simulink model "gm_minutiaeextraction_21821"  (R2018b)
(part 6 of 7)

  t38/53 -> concatenate/4789
  t38/54 -> concatenate/4790
  t38/55 -> concatenate/4791
  t38/56 -> concatenate/4792
  t38/57 -> concatenate/4793
  t38/58 -> concatenate/4794
  t38/59 -> concatenate/4795
  t38/60 -> concatenate/4796
  t38/61 -> concatenate/4797
  t38/62 -> concatenate/4798
  t38/63 -> concatenate/4799
  t38/64 -> concatenate/4800
  t38/65 -> concatenate/4801
  t38/66 -> concatenate/4802
  t38/67 -> concatenate/4803
  t38/68 -> concatenate/4804
  t38/69 -> concatenate/4805
  t38/70 -> concatenate/4806
  t38/71 -> concatenate/4807
  t38/72 -> concatenate/4808
  t38/73 -> concatenate/4809
  t38/74 -> concatenate/4810
  t38/75 -> concatenate/4811
  t38/76 -> concatenate/4812
  t38/77 -> concatenate/4813
  t38/78 -> concatenate/4814
  t38/79 -> concatenate/4815
  t38/80 -> concatenate/4816
  t38/81 -> concatenate/4817
  t38/82 -> concatenate/4818
  t38/83 -> concatenate/4819
  t38/84 -> concatenate/4820
  t38/85 -> concatenate/4821
  t38/86 -> concatenate/4822
  t38/87 -> concatenate/4823
  t38/88 -> concatenate/4824
  t38/89 -> concatenate/4825
  t38/90 -> concatenate/4826
  t38/91 -> concatenate/4827
  t38/92 -> concatenate/4828
  t38/93 -> concatenate/4829
  t38/94 -> concatenate/4830
  t38/95 -> concatenate/4831
  t38/96 -> concatenate/4832
  t38/97 -> concatenate/4833
  t38/98 -> concatenate/4834
  t38/99 -> concatenate/4835
  t38/100 -> concatenate/4836
  t38/101 -> concatenate/4837
  t38/102 -> concatenate/4838
  t38/103 -> concatenate/4839
  t38/104 -> concatenate/4840
  t38/105 -> concatenate/4841
  t38/106 -> concatenate/4842
  t38/107 -> concatenate/4843
  t38/108 -> concatenate/4844
  t38/109 -> concatenate/4845
  t38/110 -> concatenate/4846
  t38/111 -> concatenate/4847
  t38/112 -> concatenate/4848
  t38/113 -> concatenate/4849
  t38/114 -> concatenate/4850
  t38/115 -> concatenate/4851
  t38/116 -> concatenate/4852
  t38/117 -> concatenate/4853
  t38/118 -> concatenate/4854
  t38/119 -> concatenate/4855
  t38/120 -> concatenate/4856
  t38/121 -> concatenate/4857
  t38/122 -> concatenate/4858
  t38/123 -> concatenate/4859
  t38/124 -> concatenate/4860
  t38/125 -> concatenate/4861
  t38/126 -> concatenate/4862
  t38/127 -> concatenate/4863
  t38/128 -> concatenate/4864
  t39/1 -> concatenate/4865
  t39/2 -> concatenate/4866
  t39/3 -> concatenate/4867
  t39/4 -> concatenate/4868
  t39/5 -> concatenate/4869
  t39/6 -> concatenate/4870
  t39/7 -> concatenate/4871
  t39/8 -> concatenate/4872
  t39/9 -> concatenate/4873
  t39/10 -> concatenate/4874
  t39/11 -> concatenate/4875
  t39/12 -> concatenate/4876
  t39/13 -> concatenate/4877
  t39/14 -> concatenate/4878
  t39/15 -> concatenate/4879
  t39/16 -> concatenate/4880
  t39/17 -> concatenate/4881
  t39/18 -> concatenate/4882
  t39/19 -> concatenate/4883
  t39/20 -> concatenate/4884
  t39/21 -> concatenate/4885
  t39/22 -> concatenate/4886
  t39/23 -> concatenate/4887
  t39/24 -> concatenate/4888
  t39/25 -> concatenate/4889
  t39/26 -> concatenate/4890
  t39/27 -> concatenate/4891
  t39/28 -> concatenate/4892
  t39/29 -> concatenate/4893
  t39/30 -> concatenate/4894
  t39/31 -> concatenate/4895
  t39/32 -> concatenate/4896
  t39/33 -> concatenate/4897
  t39/34 -> concatenate/4898
  t39/35 -> concatenate/4899
  t39/36 -> concatenate/4900
  t39/37 -> concatenate/4901
  t39/38 -> concatenate/4902
  t39/39 -> concatenate/4903
  t39/40 -> concatenate/4904
  t39/41 -> concatenate/4905
  t39/42 -> concatenate/4906
  t39/43 -> concatenate/4907
  t39/44 -> concatenate/4908
  t39/45 -> concatenate/4909
  t39/46 -> concatenate/4910
  t39/47 -> concatenate/4911
  t39/48 -> concatenate/4912
  t39/49 -> concatenate/4913
  t39/50 -> concatenate/4914
  t39/51 -> concatenate/4915
  t39/52 -> concatenate/4916
  t39/53 -> concatenate/4917
  t39/54 -> concatenate/4918
  t39/55 -> concatenate/4919
  t39/56 -> concatenate/4920
  t39/57 -> concatenate/4921
  t39/58 -> concatenate/4922
  t39/59 -> concatenate/4923
  t39/60 -> concatenate/4924
  t39/61 -> concatenate/4925
  t39/62 -> concatenate/4926
  t39/63 -> concatenate/4927
  t39/64 -> concatenate/4928
  t39/65 -> concatenate/4929
  t39/66 -> concatenate/4930
  t39/67 -> concatenate/4931
  t39/68 -> concatenate/4932
  t39/69 -> concatenate/4933
  t39/70 -> concatenate/4934
  t39/71 -> concatenate/4935
  t39/72 -> concatenate/4936
  t39/73 -> concatenate/4937
  t39/74 -> concatenate/4938
  t39/75 -> concatenate/4939
  t39/76 -> concatenate/4940
  t39/77 -> concatenate/4941
  t39/78 -> concatenate/4942
  t39/79 -> concatenate/4943
  t39/80 -> concatenate/4944
  t39/81 -> concatenate/4945
  t39/82 -> concatenate/4946
  t39/83 -> concatenate/4947
  t39/84 -> concatenate/4948
  t39/85 -> concatenate/4949
  t39/86 -> concatenate/4950
  t39/87 -> concatenate/4951
  t39/88 -> concatenate/4952
  t39/89 -> concatenate/4953
  t39/90 -> concatenate/4954
  t39/91 -> concatenate/4955
  t39/92 -> concatenate/4956
  t39/93 -> concatenate/4957
  t39/94 -> concatenate/4958
  t39/95 -> concatenate/4959
  t39/96 -> concatenate/4960
  t39/97 -> concatenate/4961
  t39/98 -> concatenate/4962
  t39/99 -> concatenate/4963
  t39/100 -> concatenate/4964
  t39/101 -> concatenate/4965
  t39/102 -> concatenate/4966
  t39/103 -> concatenate/4967
  t39/104 -> concatenate/4968
  t39/105 -> concatenate/4969
  t39/106 -> concatenate/4970
  t39/107 -> concatenate/4971
  t39/108 -> concatenate/4972
  t39/109 -> concatenate/4973
  t39/110 -> concatenate/4974
  t39/111 -> concatenate/4975
  t39/112 -> concatenate/4976
  t39/113 -> concatenate/4977
  t39/114 -> concatenate/4978
  t39/115 -> concatenate/4979
  t39/116 -> concatenate/4980
  t39/117 -> concatenate/4981
  t39/118 -> concatenate/4982
  t39/119 -> concatenate/4983
  t39/120 -> concatenate/4984
  t39/121 -> concatenate/4985
  t39/122 -> concatenate/4986
  t39/123 -> concatenate/4987
  t39/124 -> concatenate/4988
  t39/125 -> concatenate/4989
  t39/126 -> concatenate/4990
  t39/127 -> concatenate/4991
  t39/128 -> concatenate/4992
  t40/1 -> concatenate/4993
  t40/2 -> concatenate/4994
  t40/3 -> concatenate/4995
  t40/4 -> concatenate/4996
  t40/5 -> concatenate/4997
  t40/6 -> concatenate/4998
  t40/7 -> concatenate/4999
  t40/8 -> concatenate/5000
  t40/9 -> concatenate/5001
  t40/10 -> concatenate/5002
  t40/11 -> concatenate/5003
  t40/12 -> concatenate/5004
  t40/13 -> concatenate/5005
  t40/14 -> concatenate/5006
  t40/15 -> concatenate/5007
  t40/16 -> concatenate/5008
  t40/17 -> concatenate/5009
  t40/18 -> concatenate/5010
  t40/19 -> concatenate/5011
  t40/20 -> concatenate/5012
  t40/21 -> concatenate/5013
  t40/22 -> concatenate/5014
  t40/23 -> concatenate/5015
  t40/24 -> concatenate/5016
  t40/25 -> concatenate/5017
  t40/26 -> concatenate/5018
  t40/27 -> concatenate/5019
  t40/28 -> concatenate/5020
  t40/29 -> concatenate/5021
  t40/30 -> concatenate/5022
  t40/31 -> concatenate/5023
  t40/32 -> concatenate/5024
  t40/33 -> concatenate/5025
  t40/34 -> concatenate/5026
  t40/35 -> concatenate/5027
  t40/36 -> concatenate/5028
  t40/37 -> concatenate/5029
  t40/38 -> concatenate/5030
  t40/39 -> concatenate/5031
  t40/40 -> concatenate/5032
  t40/41 -> concatenate/5033
  t40/42 -> concatenate/5034
  t40/43 -> concatenate/5035
  t40/44 -> concatenate/5036
  t40/45 -> concatenate/5037
  t40/46 -> concatenate/5038
  t40/47 -> concatenate/5039
  t40/48 -> concatenate/5040
  t40/49 -> concatenate/5041
  t40/50 -> concatenate/5042
  t40/51 -> concatenate/5043
  t40/52 -> concatenate/5044
  t40/53 -> concatenate/5045
  t40/54 -> concatenate/5046
  t40/55 -> concatenate/5047
  t40/56 -> concatenate/5048
  t40/57 -> concatenate/5049
  t40/58 -> concatenate/5050
  t40/59 -> concatenate/5051
  t40/60 -> concatenate/5052
  t40/61 -> concatenate/5053
  t40/62 -> concatenate/5054
  t40/63 -> concatenate/5055
  t40/64 -> concatenate/5056
  t40/65 -> concatenate/5057
  t40/66 -> concatenate/5058
  t40/67 -> concatenate/5059
  t40/68 -> concatenate/5060
  t40/69 -> concatenate/5061
  t40/70 -> concatenate/5062
  t40/71 -> concatenate/5063
  t40/72 -> concatenate/5064
  t40/73 -> concatenate/5065
  t40/74 -> concatenate/5066
  t40/75 -> concatenate/5067
  t40/76 -> concatenate/5068
  t40/77 -> concatenate/5069
  t40/78 -> concatenate/5070
  t40/79 -> concatenate/5071
  t40/80 -> concatenate/5072
  t40/81 -> concatenate/5073
  t40/82 -> concatenate/5074
  t40/83 -> concatenate/5075
  t40/84 -> concatenate/5076
  t40/85 -> concatenate/5077
  t40/86 -> concatenate/5078
  t40/87 -> concatenate/5079
  t40/88 -> concatenate/5080
  t40/89 -> concatenate/5081
  t40/90 -> concatenate/5082
  t40/91 -> concatenate/5083
  t40/92 -> concatenate/5084
  t40/93 -> concatenate/5085
  t40/94 -> concatenate/5086
  t40/95 -> concatenate/5087
  t40/96 -> concatenate/5088
  t40/97 -> concatenate/5089
  t40/98 -> concatenate/5090
  t40/99 -> concatenate/5091
  t40/100 -> concatenate/5092
  t40/101 -> concatenate/5093
  t40/102 -> concatenate/5094
  t40/103 -> concatenate/5095
  t40/104 -> concatenate/5096
  t40/105 -> concatenate/5097
  t40/106 -> concatenate/5098
  t40/107 -> concatenate/5099
  t40/108 -> concatenate/5100
  t40/109 -> concatenate/5101
  t40/110 -> concatenate/5102
  t40/111 -> concatenate/5103
  t40/112 -> concatenate/5104
  t40/113 -> concatenate/5105
  t40/114 -> concatenate/5106
  t40/115 -> concatenate/5107
  t40/116 -> concatenate/5108
  t40/117 -> concatenate/5109
  t40/118 -> concatenate/5110
  t40/119 -> concatenate/5111
  t40/120 -> concatenate/5112
  t40/121 -> concatenate/5113
  t40/122 -> concatenate/5114
  t40/123 -> concatenate/5115
  t40/124 -> concatenate/5116
  t40/125 -> concatenate/5117
  t40/126 -> concatenate/5118
  t40/127 -> concatenate/5119
  t40/128 -> concatenate/5120
  t41/1 -> concatenate/5121
  t41/2 -> concatenate/5122
  t41/3 -> concatenate/5123
  t41/4 -> concatenate/5124
  t41/5 -> concatenate/5125
  t41/6 -> concatenate/5126
  t41/7 -> concatenate/5127
  t41/8 -> concatenate/5128
  t41/9 -> concatenate/5129
  t41/10 -> concatenate/5130
  t41/11 -> concatenate/5131
  t41/12 -> concatenate/5132
  t41/13 -> concatenate/5133
  t41/14 -> concatenate/5134
  t41/15 -> concatenate/5135
  t41/16 -> concatenate/5136
  t41/17 -> concatenate/5137
  t41/18 -> concatenate/5138
  t41/19 -> concatenate/5139
  t41/20 -> concatenate/5140
  t41/21 -> concatenate/5141
  t41/22 -> concatenate/5142
  t41/23 -> concatenate/5143
  t41/24 -> concatenate/5144
  t41/25 -> concatenate/5145
  t41/26 -> concatenate/5146
  t41/27 -> concatenate/5147
  t41/28 -> concatenate/5148
  t41/29 -> concatenate/5149
  t41/30 -> concatenate/5150
  t41/31 -> concatenate/5151
  t41/32 -> concatenate/5152
  t41/33 -> concatenate/5153
  t41/34 -> concatenate/5154
  t41/35 -> concatenate/5155
  t41/36 -> concatenate/5156
  t41/37 -> concatenate/5157
  t41/38 -> concatenate/5158
  t41/39 -> concatenate/5159
  t41/40 -> concatenate/5160
  t41/41 -> concatenate/5161
  t41/42 -> concatenate/5162
  t41/43 -> concatenate/5163
  t41/44 -> concatenate/5164
  t41/45 -> concatenate/5165
  t41/46 -> concatenate/5166
  t41/47 -> concatenate/5167
  t41/48 -> concatenate/5168
  t41/49 -> concatenate/5169
  t41/50 -> concatenate/5170
  t41/51 -> concatenate/5171
  t41/52 -> concatenate/5172
  t41/53 -> concatenate/5173
  t41/54 -> concatenate/5174
  t41/55 -> concatenate/5175
  t41/56 -> concatenate/5176
  t41/57 -> concatenate/5177
  t41/58 -> concatenate/5178
  t41/59 -> concatenate/5179
  t41/60 -> concatenate/5180
  t41/61 -> concatenate/5181
  t41/62 -> concatenate/5182
  t41/63 -> concatenate/5183
  t41/64 -> concatenate/5184
  t41/65 -> concatenate/5185
  t41/66 -> concatenate/5186
  t41/67 -> concatenate/5187
  t41/68 -> concatenate/5188
  t41/69 -> concatenate/5189
  t41/70 -> concatenate/5190
  t41/71 -> concatenate/5191
  t41/72 -> concatenate/5192
  t41/73 -> concatenate/5193
  t41/74 -> concatenate/5194
  t41/75 -> concatenate/5195
  t41/76 -> concatenate/5196
  t41/77 -> concatenate/5197
  t41/78 -> concatenate/5198
  t41/79 -> concatenate/5199
  t41/80 -> concatenate/5200
  t41/81 -> concatenate/5201
  t41/82 -> concatenate/5202
  t41/83 -> concatenate/5203
  t41/84 -> concatenate/5204
  t41/85 -> concatenate/5205
  t41/86 -> concatenate/5206
  t41/87 -> concatenate/5207
  t41/88 -> concatenate/5208
  t41/89 -> concatenate/5209
  t41/90 -> concatenate/5210
  t41/91 -> concatenate/5211
  t41/92 -> concatenate/5212
  t41/93 -> concatenate/5213
  t41/94 -> concatenate/5214
  t41/95 -> concatenate/5215
  t41/96 -> concatenate/5216
  t41/97 -> concatenate/5217
  t41/98 -> concatenate/5218
  t41/99 -> concatenate/5219
  t41/100 -> concatenate/5220
  t41/101 -> concatenate/5221
  t41/102 -> concatenate/5222
  t41/103 -> concatenate/5223
  t41/104 -> concatenate/5224
  t41/105 -> concatenate/5225
  t41/106 -> concatenate/5226
  t41/107 -> concatenate/5227
  t41/108 -> concatenate/5228
  t41/109 -> concatenate/5229
  t41/110 -> concatenate/5230
  t41/111 -> concatenate/5231
  t41/112 -> concatenate/5232
  t41/113 -> concatenate/5233
  t41/114 -> concatenate/5234
  t41/115 -> concatenate/5235
  t41/116 -> concatenate/5236
  t41/117 -> concatenate/5237
  t41/118 -> concatenate/5238
  t41/119 -> concatenate/5239
  t41/120 -> concatenate/5240
  t41/121 -> concatenate/5241
  t41/122 -> concatenate/5242
  t41/123 -> concatenate/5243
  t41/124 -> concatenate/5244
  t41/125 -> concatenate/5245
  t41/126 -> concatenate/5246
  t41/127 -> concatenate/5247
  t41/128 -> concatenate/5248
  t42/1 -> concatenate/5249
  t42/2 -> concatenate/5250
  t42/3 -> concatenate/5251
  t42/4 -> concatenate/5252
  t42/5 -> concatenate/5253
  t42/6 -> concatenate/5254
  t42/7 -> concatenate/5255
  t42/8 -> concatenate/5256
  t42/9 -> concatenate/5257
  t42/10 -> concatenate/5258
  t42/11 -> concatenate/5259
  t42/12 -> concatenate/5260
  t42/13 -> concatenate/5261
  t42/14 -> concatenate/5262
  t42/15 -> concatenate/5263
  t42/16 -> concatenate/5264
  t42/17 -> concatenate/5265
  t42/18 -> concatenate/5266
  t42/19 -> concatenate/5267
  t42/20 -> concatenate/5268
  t42/21 -> concatenate/5269
  t42/22 -> concatenate/5270
  t42/23 -> concatenate/5271
  t42/24 -> concatenate/5272
  t42/25 -> concatenate/5273
  t42/26 -> concatenate/5274
  t42/27 -> concatenate/5275
  t42/28 -> concatenate/5276
  t42/29 -> concatenate/5277
  t42/30 -> concatenate/5278
  t42/31 -> concatenate/5279
  t42/32 -> concatenate/5280
  t42/33 -> concatenate/5281
  t42/34 -> concatenate/5282
  t42/35 -> concatenate/5283
  t42/36 -> concatenate/5284
  t42/37 -> concatenate/5285
  t42/38 -> concatenate/5286
  t42/39 -> concatenate/5287
  t42/40 -> concatenate/5288
  t42/41 -> concatenate/5289
  t42/42 -> concatenate/5290
  t42/43 -> concatenate/5291
  t42/44 -> concatenate/5292
  t42/45 -> concatenate/5293
  t42/46 -> concatenate/5294
  t42/47 -> concatenate/5295
  t42/48 -> concatenate/5296
  t42/49 -> concatenate/5297
  t42/50 -> concatenate/5298
  t42/51 -> concatenate/5299
  t42/52 -> concatenate/5300
  t42/53 -> concatenate/5301
  t42/54 -> concatenate/5302
  t42/55 -> concatenate/5303
  t42/56 -> concatenate/5304
  t42/57 -> concatenate/5305
  t42/58 -> concatenate/5306
  t42/59 -> concatenate/5307
  t42/60 -> concatenate/5308
  t42/61 -> concatenate/5309
  t42/62 -> concatenate/5310
  t42/63 -> concatenate/5311
  t42/64 -> concatenate/5312
  t42/65 -> concatenate/5313
  t42/66 -> concatenate/5314
  t42/67 -> concatenate/5315
  t42/68 -> concatenate/5316
  t42/69 -> concatenate/5317
  t42/70 -> concatenate/5318
  t42/71 -> concatenate/5319
  t42/72 -> concatenate/5320
  t42/73 -> concatenate/5321
  t42/74 -> concatenate/5322
  t42/75 -> concatenate/5323
  t42/76 -> concatenate/5324
  t42/77 -> concatenate/5325
  t42/78 -> concatenate/5326
  t42/79 -> concatenate/5327
  t42/80 -> concatenate/5328
  t42/81 -> concatenate/5329
  t42/82 -> concatenate/5330
  t42/83 -> concatenate/5331
  t42/84 -> concatenate/5332
  t42/85 -> concatenate/5333
  t42/86 -> concatenate/5334
  t42/87 -> concatenate/5335
  t42/88 -> concatenate/5336
  t42/89 -> concatenate/5337
  t42/90 -> concatenate/5338
  t42/91 -> concatenate/5339
  t42/92 -> concatenate/5340
  t42/93 -> concatenate/5341
  t42/94 -> concatenate/5342
  t42/95 -> concatenate/5343
  t42/96 -> concatenate/5344
  t42/97 -> concatenate/5345
  t42/98 -> concatenate/5346
  t42/99 -> concatenate/5347
  t42/100 -> concatenate/5348
  t42/101 -> concatenate/5349
  t42/102 -> concatenate/5350
  t42/103 -> concatenate/5351
  t42/104 -> concatenate/5352
  t42/105 -> concatenate/5353
  t42/106 -> concatenate/5354
  t42/107 -> concatenate/5355
  t42/108 -> concatenate/5356
  t42/109 -> concatenate/5357
  t42/110 -> concatenate/5358
  t42/111 -> concatenate/5359
  t42/112 -> concatenate/5360
  t42/113 -> concatenate/5361
  t42/114 -> concatenate/5362
  t42/115 -> concatenate/5363
  t42/116 -> concatenate/5364
  t42/117 -> concatenate/5365
  t42/118 -> concatenate/5366
  t42/119 -> concatenate/5367
  t42/120 -> concatenate/5368
  t42/121 -> concatenate/5369
  t42/122 -> concatenate/5370
  t42/123 -> concatenate/5371
  t42/124 -> concatenate/5372
  t42/125 -> concatenate/5373
  t42/126 -> concatenate/5374
  t42/127 -> concatenate/5375
  t42/128 -> concatenate/5376
  t43/1 -> concatenate/5377
  t43/2 -> concatenate/5378
  t43/3 -> concatenate/5379
  t43/4 -> concatenate/5380
  t43/5 -> concatenate/5381
  t43/6 -> concatenate/5382
  t43/7 -> concatenate/5383
  t43/8 -> concatenate/5384
  t43/9 -> concatenate/5385
  t43/10 -> concatenate/5386
  t43/11 -> concatenate/5387
  t43/12 -> concatenate/5388
  t43/13 -> concatenate/5389
  t43/14 -> concatenate/5390
  t43/15 -> concatenate/5391
  t43/16 -> concatenate/5392
  t43/17 -> concatenate/5393
  t43/18 -> concatenate/5394
  t43/19 -> concatenate/5395
  t43/20 -> concatenate/5396
  t43/21 -> concatenate/5397
  t43/22 -> concatenate/5398
  t43/23 -> concatenate/5399
  t43/24 -> concatenate/5400
  t43/25 -> concatenate/5401
  t43/26 -> concatenate/5402
  t43/27 -> concatenate/5403
  t43/28 -> concatenate/5404
  t43/29 -> concatenate/5405
  t43/30 -> concatenate/5406
  t43/31 -> concatenate/5407
  t43/32 -> concatenate/5408
  t43/33 -> concatenate/5409
  t43/34 -> concatenate/5410
  t43/35 -> concatenate/5411
  t43/36 -> concatenate/5412
  t43/37 -> concatenate/5413
  t43/38 -> concatenate/5414
  t43/39 -> concatenate/5415
  t43/40 -> concatenate/5416
  t43/41 -> concatenate/5417
  t43/42 -> concatenate/5418
  t43/43 -> concatenate/5419
  t43/44 -> concatenate/5420
  t43/45 -> concatenate/5421
  t43/46 -> concatenate/5422
  t43/47 -> concatenate/5423
  t43/48 -> concatenate/5424
  t43/49 -> concatenate/5425
  t43/50 -> concatenate/5426
  t43/51 -> concatenate/5427
  t43/52 -> concatenate/5428
  t43/53 -> concatenate/5429
  t43/54 -> concatenate/5430
  t43/55 -> concatenate/5431
  t43/56 -> concatenate/5432
  t43/57 -> concatenate/5433
  t43/58 -> concatenate/5434
  t43/59 -> concatenate/5435
  t43/60 -> concatenate/5436
  t43/61 -> concatenate/5437
  t43/62 -> concatenate/5438
  t43/63 -> concatenate/5439
  t43/64 -> concatenate/5440
  t43/65 -> concatenate/5441
  t43/66 -> concatenate/5442
  t43/67 -> concatenate/5443
  t43/68 -> concatenate/5444
  t43/69 -> concatenate/5445
  t43/70 -> concatenate/5446
  t43/71 -> concatenate/5447
  t43/72 -> concatenate/5448
  t43/73 -> concatenate/5449
  t43/74 -> concatenate/5450
  t43/75 -> concatenate/5451
  t43/76 -> concatenate/5452
  t43/77 -> concatenate/5453
  t43/78 -> concatenate/5454
  t43/79 -> concatenate/5455
  t43/80 -> concatenate/5456
  t43/81 -> concatenate/5457
  t43/82 -> concatenate/5458
  t43/83 -> concatenate/5459
  t43/84 -> concatenate/5460
  t43/85 -> concatenate/5461
  t43/86 -> concatenate/5462
  t43/87 -> concatenate/5463
  t43/88 -> concatenate/5464
  t43/89 -> concatenate/5465
  t43/90 -> concatenate/5466
  t43/91 -> concatenate/5467
  t43/92 -> concatenate/5468
  t43/93 -> concatenate/5469
  t43/94 -> concatenate/5470
  t43/95 -> concatenate/5471
  t43/96 -> concatenate/5472
  t43/97 -> concatenate/5473
  t43/98 -> concatenate/5474
  t43/99 -> concatenate/5475
  t43/100 -> concatenate/5476
  t43/101 -> concatenate/5477
  t43/102 -> concatenate/5478
  t43/103 -> concatenate/5479
  t43/104 -> concatenate/5480
  t43/105 -> concatenate/5481
  t43/106 -> concatenate/5482
  t43/107 -> concatenate/5483
  t43/108 -> concatenate/5484
  t43/109 -> concatenate/5485
  t43/110 -> concatenate/5486
  t43/111 -> concatenate/5487
  t43/112 -> concatenate/5488
  t43/113 -> concatenate/5489
  t43/114 -> concatenate/5490
  t43/115 -> concatenate/5491
  t43/116 -> concatenate/5492
  t43/117 -> concatenate/5493
  t43/118 -> concatenate/5494
  t43/119 -> concatenate/5495
  t43/120 -> concatenate/5496
  t43/121 -> concatenate/5497
  t43/122 -> concatenate/5498
  t43/123 -> concatenate/5499
  t43/124 -> concatenate/5500
  t43/125 -> concatenate/5501
  t43/126 -> concatenate/5502
  t43/127 -> concatenate/5503
  t43/128 -> concatenate/5504
  t44/1 -> concatenate/5505
  t44/2 -> concatenate/5506
  t44/3 -> concatenate/5507
  t44/4 -> concatenate/5508
  t44/5 -> concatenate/5509
  t44/6 -> concatenate/5510
  t44/7 -> concatenate/5511
  t44/8 -> concatenate/5512
  t44/9 -> concatenate/5513
  t44/10 -> concatenate/5514
  t44/11 -> concatenate/5515
  t44/12 -> concatenate/5516
  t44/13 -> concatenate/5517
  t44/14 -> concatenate/5518
  t44/15 -> concatenate/5519
  t44/16 -> concatenate/5520
  t44/17 -> concatenate/5521
  t44/18 -> concatenate/5522
  t44/19 -> concatenate/5523
  t44/20 -> concatenate/5524
  t44/21 -> concatenate/5525
  t44/22 -> concatenate/5526
  t44/23 -> concatenate/5527
  t44/24 -> concatenate/5528
  t44/25 -> concatenate/5529
  t44/26 -> concatenate/5530
  t44/27 -> concatenate/5531
  t44/28 -> concatenate/5532
  t44/29 -> concatenate/5533
  t44/30 -> concatenate/5534
  t44/31 -> concatenate/5535
  t44/32 -> concatenate/5536
  t44/33 -> concatenate/5537
  t44/34 -> concatenate/5538
  t44/35 -> concatenate/5539
  t44/36 -> concatenate/5540
  t44/37 -> concatenate/5541
  t44/38 -> concatenate/5542
  t44/39 -> concatenate/5543
  t44/40 -> concatenate/5544
  t44/41 -> concatenate/5545
  t44/42 -> concatenate/5546
  t44/43 -> concatenate/5547
  t44/44 -> concatenate/5548
  t44/45 -> concatenate/5549
  t44/46 -> concatenate/5550
  t44/47 -> concatenate/5551
  t44/48 -> concatenate/5552
  t44/49 -> concatenate/5553
  t44/50 -> concatenate/5554
  t44/51 -> concatenate/5555
  t44/52 -> concatenate/5556
  t44/53 -> concatenate/5557
  t44/54 -> concatenate/5558
  t44/55 -> concatenate/5559
  t44/56 -> concatenate/5560
  t44/57 -> concatenate/5561
  t44/58 -> concatenate/5562
  t44/59 -> concatenate/5563
  t44/60 -> concatenate/5564
  t44/61 -> concatenate/5565
  t44/62 -> concatenate/5566
  t44/63 -> concatenate/5567
  t44/64 -> concatenate/5568
  t44/65 -> concatenate/5569
  t44/66 -> concatenate/5570
  t44/67 -> concatenate/5571
  t44/68 -> concatenate/5572
  t44/69 -> concatenate/5573
  t44/70 -> concatenate/5574
  t44/71 -> concatenate/5575
  t44/72 -> concatenate/5576
  t44/73 -> concatenate/5577
  t44/74 -> concatenate/5578
  t44/75 -> concatenate/5579
  t44/76 -> concatenate/5580
  t44/77 -> concatenate/5581
  t44/78 -> concatenate/5582
  t44/79 -> concatenate/5583
  t44/80 -> concatenate/5584
  t44/81 -> concatenate/5585
  t44/82 -> concatenate/5586
  t44/83 -> concatenate/5587
  t44/84 -> concatenate/5588
  t44/85 -> concatenate/5589
  t44/86 -> concatenate/5590
  t44/87 -> concatenate/5591
  t44/88 -> concatenate/5592
  t44/89 -> concatenate/5593
  t44/90 -> concatenate/5594
  t44/91 -> concatenate/5595
  t44/92 -> concatenate/5596
  t44/93 -> concatenate/5597
  t44/94 -> concatenate/5598
  t44/95 -> concatenate/5599
  t44/96 -> concatenate/5600
  t44/97 -> concatenate/5601
  t44/98 -> concatenate/5602
  t44/99 -> concatenate/5603
  t44/100 -> concatenate/5604
  t44/101 -> concatenate/5605
  t44/102 -> concatenate/5606
  t44/103 -> concatenate/5607
  t44/104 -> concatenate/5608
  t44/105 -> concatenate/5609
  t44/106 -> concatenate/5610
  t44/107 -> concatenate/5611
  t44/108 -> concatenate/5612
  t44/109 -> concatenate/5613
  t44/110 -> concatenate/5614
  t44/111 -> concatenate/5615
  t44/112 -> concatenate/5616
  t44/113 -> concatenate/5617
  t44/114 -> concatenate/5618
  t44/115 -> concatenate/5619
  t44/116 -> concatenate/5620
  t44/117 -> concatenate/5621
  t44/118 -> concatenate/5622
  t44/119 -> concatenate/5623
  t44/120 -> concatenate/5624
  t44/121 -> concatenate/5625
  t44/122 -> concatenate/5626
  t44/123 -> concatenate/5627
  t44/124 -> concatenate/5628
  t44/125 -> concatenate/5629
  t44/126 -> concatenate/5630
  t44/127 -> concatenate/5631
  t44/128 -> concatenate/5632
  t45/1 -> concatenate/5633
  t45/2 -> concatenate/5634
  t45/3 -> concatenate/5635
  t45/4 -> concatenate/5636
  t45/5 -> concatenate/5637
  t45/6 -> concatenate/5638
  t45/7 -> concatenate/5639
  t45/8 -> concatenate/5640
  t45/9 -> concatenate/5641
  t45/10 -> concatenate/5642
  t45/11 -> concatenate/5643
  t45/12 -> concatenate/5644
  t45/13 -> concatenate/5645
  t45/14 -> concatenate/5646
  t45/15 -> concatenate/5647
  t45/16 -> concatenate/5648
  t45/17 -> concatenate/5649
  t45/18 -> concatenate/5650
  t45/19 -> concatenate/5651
  t45/20 -> concatenate/5652
  t45/21 -> concatenate/5653
  t45/22 -> concatenate/5654
  t45/23 -> concatenate/5655
  t45/24 -> concatenate/5656
  t45/25 -> concatenate/5657
  t45/26 -> concatenate/5658
  t45/27 -> concatenate/5659
  t45/28 -> concatenate/5660
  t45/29 -> concatenate/5661
  t45/30 -> concatenate/5662
  t45/31 -> concatenate/5663
  t45/32 -> concatenate/5664
  t45/33 -> concatenate/5665
  t45/34 -> concatenate/5666
  t45/35 -> concatenate/5667
  t45/36 -> concatenate/5668
  t45/37 -> concatenate/5669
  t45/38 -> concatenate/5670
  t45/39 -> concatenate/5671
  t45/40 -> concatenate/5672
  t45/41 -> concatenate/5673
  t45/42 -> concatenate/5674
  t45/43 -> concatenate/5675
  t45/44 -> concatenate/5676
  t45/45 -> concatenate/5677
  t45/46 -> concatenate/5678
  t45/47 -> concatenate/5679
  t45/48 -> concatenate/5680
  t45/49 -> concatenate/5681
  t45/50 -> concatenate/5682
  t45/51 -> concatenate/5683
  t45/52 -> concatenate/5684
  t45/53 -> concatenate/5685
  t45/54 -> concatenate/5686
  t45/55 -> concatenate/5687
  t45/56 -> concatenate/5688
  t45/57 -> concatenate/5689
  t45/58 -> concatenate/5690
  t45/59 -> concatenate/5691
  t45/60 -> concatenate/5692
  t45/61 -> concatenate/5693
  t45/62 -> concatenate/5694
  t45/63 -> concatenate/5695
  t45/64 -> concatenate/5696
  t45/65 -> concatenate/5697
  t45/66 -> concatenate/5698
  t45/67 -> concatenate/5699
  t45/68 -> concatenate/5700
  t45/69 -> concatenate/5701
  t45/70 -> concatenate/5702
  t45/71 -> concatenate/5703
  t45/72 -> concatenate/5704
  t45/73 -> concatenate/5705
  t45/74 -> concatenate/5706
  t45/75 -> concatenate/5707
  t45/76 -> concatenate/5708
  t45/77 -> concatenate/5709
  t45/78 -> concatenate/5710
  t45/79 -> concatenate/5711
  t45/80 -> concatenate/5712
  t45/81 -> concatenate/5713
  t45/82 -> concatenate/5714
  t45/83 -> concatenate/5715
  t45/84 -> concatenate/5716
  t45/85 -> concatenate/5717
  t45/86 -> concatenate/5718
  t45/87 -> concatenate/5719
  t45/88 -> concatenate/5720
  t45/89 -> concatenate/5721
  t45/90 -> concatenate/5722
  t45/91 -> concatenate/5723
  t45/92 -> concatenate/5724
  t45/93 -> concatenate/5725
  t45/94 -> concatenate/5726
  t45/95 -> concatenate/5727
  t45/96 -> concatenate/5728
  t45/97 -> concatenate/5729
  t45/98 -> concatenate/5730
  t45/99 -> concatenate/5731
  t45/100 -> concatenate/5732
  t45/101 -> concatenate/5733
  t45/102 -> concatenate/5734
  t45/103 -> concatenate/5735
  t45/104 -> concatenate/5736
  t45/105 -> concatenate/5737
  t45/106 -> concatenate/5738
  t45/107 -> concatenate/5739
  t45/108 -> concatenate/5740
  t45/109 -> concatenate/5741
  t45/110 -> concatenate/5742
  t45/111 -> concatenate/5743
  t45/112 -> concatenate/5744
  t45/113 -> concatenate/5745
  t45/114 -> concatenate/5746
  t45/115 -> concatenate/5747
  t45/116 -> concatenate/5748
  t45/117 -> concatenate/5749
  t45/118 -> concatenate/5750
  t45/119 -> concatenate/5751
  t45/120 -> concatenate/5752
  t45/121 -> concatenate/5753
  t45/122 -> concatenate/5754
  t45/123 -> concatenate/5755
  t45/124 -> concatenate/5756
  t45/125 -> concatenate/5757
  t45/126 -> concatenate/5758
  t45/127 -> concatenate/5759
  t45/128 -> concatenate/5760
  t46/1 -> concatenate/5761
  t46/2 -> concatenate/5762
  t46/3 -> concatenate/5763
  t46/4 -> concatenate/5764
  t46/5 -> concatenate/5765
  t46/6 -> concatenate/5766
  t46/7 -> concatenate/5767
  t46/8 -> concatenate/5768
  t46/9 -> concatenate/5769
  t46/10 -> concatenate/5770
  t46/11 -> concatenate/5771
  t46/12 -> concatenate/5772
  t46/13 -> concatenate/5773
  t46/14 -> concatenate/5774
  t46/15 -> concatenate/5775
  t46/16 -> concatenate/5776
  t46/17 -> concatenate/5777
  t46/18 -> concatenate/5778
  t46/19 -> concatenate/5779
  t46/20 -> concatenate/5780
  t46/21 -> concatenate/5781
  t46/22 -> concatenate/5782
  t46/23 -> concatenate/5783
  t46/24 -> concatenate/5784
  t46/25 -> concatenate/5785
  t46/26 -> concatenate/5786
  t46/27 -> concatenate/5787
  t46/28 -> concatenate/5788
  t46/29 -> concatenate/5789
  t46/30 -> concatenate/5790
  t46/31 -> concatenate/5791
  t46/32 -> concatenate/5792
  t46/33 -> concatenate/5793
  t46/34 -> concatenate/5794
  t46/35 -> concatenate/5795
  t46/36 -> concatenate/5796
  t46/37 -> concatenate/5797
  t46/38 -> concatenate/5798
  t46/39 -> concatenate/5799
  t46/40 -> concatenate/5800
  t46/41 -> concatenate/5801
  t46/42 -> concatenate/5802
  t46/43 -> concatenate/5803
  t46/44 -> concatenate/5804
  t46/45 -> concatenate/5805
  t46/46 -> concatenate/5806
  t46/47 -> concatenate/5807
  t46/48 -> concatenate/5808
  t46/49 -> concatenate/5809
  t46/50 -> concatenate/5810
  t46/51 -> concatenate/5811
  t46/52 -> concatenate/5812
  t46/53 -> concatenate/5813
  t46/54 -> concatenate/5814
  t46/55 -> concatenate/5815
  t46/56 -> concatenate/5816
  t46/57 -> concatenate/5817
  t46/58 -> concatenate/5818
  t46/59 -> concatenate/5819
  t46/60 -> concatenate/5820
  t46/61 -> concatenate/5821
  t46/62 -> concatenate/5822
  t46/63 -> concatenate/5823
  t46/64 -> concatenate/5824
  t46/65 -> concatenate/5825
  t46/66 -> concatenate/5826
  t46/67 -> concatenate/5827
  t46/68 -> concatenate/5828
  t46/69 -> concatenate/5829
  t46/70 -> concatenate/5830
  t46/71 -> concatenate/5831
  t46/72 -> concatenate/5832
  t46/73 -> concatenate/5833
  t46/74 -> concatenate/5834
  t46/75 -> concatenate/5835
  t46/76 -> concatenate/5836
  t46/77 -> concatenate/5837
  t46/78 -> concatenate/5838
  t46/79 -> concatenate/5839
  t46/80 -> concatenate/5840
  t46/81 -> concatenate/5841
  t46/82 -> concatenate/5842
  t46/83 -> concatenate/5843
  t46/84 -> concatenate/5844
  t46/85 -> concatenate/5845
  t46/86 -> concatenate/5846
  t46/87 -> concatenate/5847
  t46/88 -> concatenate/5848
  t46/89 -> concatenate/5849
  t46/90 -> concatenate/5850
  t46/91 -> concatenate/5851
  t46/92 -> concatenate/5852
  t46/93 -> concatenate/5853
  t46/94 -> concatenate/5854
  t46/95 -> concatenate/5855
  t46/96 -> concatenate/5856
  t46/97 -> concatenate/5857
  t46/98 -> concatenate/5858
  t46/99 -> concatenate/5859
  t46/100 -> concatenate/5860
  t46/101 -> concatenate/5861
  t46/102 -> concatenate/5862
  t46/103 -> concatenate/5863
  t46/104 -> concatenate/5864
  t46/105 -> concatenate/5865
  t46/106 -> concatenate/5866
  t46/107 -> concatenate/5867
  t46/108 -> concatenate/5868
  t46/109 -> concatenate/5869
  t46/110 -> concatenate/5870
  t46/111 -> concatenate/5871
  t46/112 -> concatenate/5872
  t46/113 -> concatenate/5873
  t46/114 -> concatenate/5874
  t46/115 -> concatenate/5875
  t46/116 -> concatenate/5876
  t46/117 -> concatenate/5877
  t46/118 -> concatenate/5878
  t46/119 -> concatenate/5879
  t46/120 -> concatenate/5880
  t46/121 -> concatenate/5881
  t46/122 -> concatenate/5882
  t46/123 -> concatenate/5883
  t46/124 -> concatenate/5884
  t46/125 -> concatenate/5885
  t46/126 -> concatenate/5886
  t46/127 -> concatenate/5887
  t46/128 -> concatenate/5888
  t47/1 -> concatenate/5889
  t47/2 -> concatenate/5890
  t47/3 -> concatenate/5891
  t47/4 -> concatenate/5892
  t47/5 -> concatenate/5893
  t47/6 -> concatenate/5894
  t47/7 -> concatenate/5895
  t47/8 -> concatenate/5896
  t47/9 -> concatenate/5897
  t47/10 -> concatenate/5898
  t47/11 -> concatenate/5899
  t47/12 -> concatenate/5900
  t47/13 -> concatenate/5901
  t47/14 -> concatenate/5902
  t47/15 -> concatenate/5903
  t47/16 -> concatenate/5904
  t47/17 -> concatenate/5905
  t47/18 -> concatenate/5906
  t47/19 -> concatenate/5907
  t47/20 -> concatenate/5908
  t47/21 -> concatenate/5909
  t47/22 -> concatenate/5910
  t47/23 -> concatenate/5911
  t47/24 -> concatenate/5912
  t47/25 -> concatenate/5913
  t47/26 -> concatenate/5914
  t47/27 -> concatenate/5915
  t47/28 -> concatenate/5916
  t47/29 -> concatenate/5917
  t47/30 -> concatenate/5918
  t47/31 -> concatenate/5919
  t47/32 -> concatenate/5920
  t47/33 -> concatenate/5921
  t47/34 -> concatenate/5922
  t47/35 -> concatenate/5923
  t47/36 -> concatenate/5924
  t47/37 -> concatenate/5925
  t47/38 -> concatenate/5926
  t47/39 -> concatenate/5927
  t47/40 -> concatenate/5928
  t47/41 -> concatenate/5929
  t47/42 -> concatenate/5930
  t47/43 -> concatenate/5931
  t47/44 -> concatenate/5932
  t47/45 -> concatenate/5933
  t47/46 -> concatenate/5934
  t47/47 -> concatenate/5935
  t47/48 -> concatenate/5936
  t47/49 -> concatenate/5937
  t47/50 -> concatenate/5938
  t47/51 -> concatenate/5939
  t47/52 -> concatenate/5940
  t47/53 -> concatenate/5941
  t47/54 -> concatenate/5942
  t47/55 -> concatenate/5943
  t47/56 -> concatenate/5944
  t47/57 -> concatenate/5945
  t47/58 -> concatenate/5946
  t47/59 -> concatenate/5947
  t47/60 -> concatenate/5948
  t47/61 -> concatenate/5949
  t47/62 -> concatenate/5950
  t47/63 -> concatenate/5951
  t47/64 -> concatenate/5952
  t47/65 -> concatenate/5953
  t47/66 -> concatenate/5954
  t47/67 -> concatenate/5955
  t47/68 -> concatenate/5956
  t47/69 -> concatenate/5957
  t47/70 -> concatenate/5958
  t47/71 -> concatenate/5959
  t47/72 -> concatenate/5960
  t47/73 -> concatenate/5961
  t47/74 -> concatenate/5962
  t47/75 -> concatenate/5963
  t47/76 -> concatenate/5964
  t47/77 -> concatenate/5965
  t47/78 -> concatenate/5966
  t47/79 -> concatenate/5967
  t47/80 -> concatenate/5968
  t47/81 -> concatenate/5969
  t47/82 -> concatenate/5970
  t47/83 -> concatenate/5971
  t47/84 -> concatenate/5972
  t47/85 -> concatenate/5973
  t47/86 -> concatenate/5974
  t47/87 -> concatenate/5975
  t47/88 -> concatenate/5976
  t47/89 -> concatenate/5977
  t47/90 -> concatenate/5978
  t47/91 -> concatenate/5979
  t47/92 -> concatenate/5980
  t47/93 -> concatenate/5981
  t47/94 -> concatenate/5982
  t47/95 -> concatenate/5983
  t47/96 -> concatenate/5984
  t47/97 -> concatenate/5985
  t47/98 -> concatenate/5986
  t47/99 -> concatenate/5987
  t47/100 -> concatenate/5988
  t47/101 -> concatenate/5989
  t47/102 -> concatenate/5990
  t47/103 -> concatenate/5991
  t47/104 -> concatenate/5992
  t47/105 -> concatenate/5993
  t47/106 -> concatenate/5994
  t47/107 -> concatenate/5995
  t47/108 -> concatenate/5996
  t47/109 -> concatenate/5997
  t47/110 -> concatenate/5998
  t47/111 -> concatenate/5999
  t47/112 -> concatenate/6000
  t47/113 -> concatenate/6001
  t47/114 -> concatenate/6002
  t47/115 -> concatenate/6003
  t47/116 -> concatenate/6004
  t47/117 -> concatenate/6005
  t47/118 -> concatenate/6006
  t47/119 -> concatenate/6007
  t47/120 -> concatenate/6008
  t47/121 -> concatenate/6009
  t47/122 -> concatenate/6010
  t47/123 -> concatenate/6011
  t47/124 -> concatenate/6012
  t47/125 -> concatenate/6013
  t47/126 -> concatenate/6014
  t47/127 -> concatenate/6015
  t47/128 -> concatenate/6016
  t48/1 -> concatenate/6017
  t48/2 -> concatenate/6018
  t48/3 -> concatenate/6019
  t48/4 -> concatenate/6020
  t48/5 -> concatenate/6021
  t48/6 -> concatenate/6022
  t48/7 -> concatenate/6023
  t48/8 -> concatenate/6024
  t48/9 -> concatenate/6025
  t48/10 -> concatenate/6026
  t48/11 -> concatenate/6027
  t48/12 -> concatenate/6028
  t48/13 -> concatenate/6029
  t48/14 -> concatenate/6030
  t48/15 -> concatenate/6031
  t48/16 -> concatenate/6032
  t48/17 -> concatenate/6033
  t48/18 -> concatenate/6034
  t48/19 -> concatenate/6035
  t48/20 -> concatenate/6036
  t48/21 -> concatenate/6037
  t48/22 -> concatenate/6038
  t48/23 -> concatenate/6039
  t48/24 -> concatenate/6040
  t48/25 -> concatenate/6041
  t48/26 -> concatenate/6042
  t48/27 -> concatenate/6043
  t48/28 -> concatenate/6044
  t48/29 -> concatenate/6045
  t48/30 -> concatenate/6046
  t48/31 -> concatenate/6047
  t48/32 -> concatenate/6048
  t48/33 -> concatenate/6049
  t48/34 -> concatenate/6050
  t48/35 -> concatenate/6051
  t48/36 -> concatenate/6052
  t48/37 -> concatenate/6053
  t48/38 -> concatenate/6054
  t48/39 -> concatenate/6055
  t48/40 -> concatenate/6056
  t48/41 -> concatenate/6057
  t48/42 -> concatenate/6058
  t48/43 -> concatenate/6059
  t48/44 -> concatenate/6060
  t48/45 -> concatenate/6061
  t48/46 -> concatenate/6062
  t48/47 -> concatenate/6063
  t48/48 -> concatenate/6064
  t48/49 -> concatenate/6065
  t48/50 -> concatenate/6066
  t48/51 -> concatenate/6067
  t48/52 -> concatenate/6068
  t48/53 -> concatenate/6069
  t48/54 -> concatenate/6070
  t48/55 -> concatenate/6071
  t48/56 -> concatenate/6072
  t48/57 -> concatenate/6073
  t48/58 -> concatenate/6074
  t48/59 -> concatenate/6075
  t48/60 -> concatenate/6076
  t48/61 -> concatenate/6077
  t48/62 -> concatenate/6078
  t48/63 -> concatenate/6079
  t48/64 -> concatenate/6080
  t48/65 -> concatenate/6081
  t48/66 -> concatenate/6082
  t48/67 -> concatenate/6083
  t48/68 -> concatenate/6084
  t48/69 -> concatenate/6085
  t48/70 -> concatenate/6086
  t48/71 -> concatenate/6087
  t48/72 -> concatenate/6088
  t48/73 -> concatenate/6089
  t48/74 -> concatenate/6090
  t48/75 -> concatenate/6091
  t48/76 -> concatenate/6092
  t48/77 -> concatenate/6093
  t48/78 -> concatenate/6094
  t48/79 -> concatenate/6095
  t48/80 -> concatenate/6096
  t48/81 -> concatenate/6097
  t48/82 -> concatenate/6098
  t48/83 -> concatenate/6099
  t48/84 -> concatenate/6100
  t48/85 -> concatenate/6101
  t48/86 -> concatenate/6102
  t48/87 -> concatenate/6103
  t48/88 -> concatenate/6104
  t48/89 -> concatenate/6105
  t48/90 -> concatenate/6106
  t48/91 -> concatenate/6107
  t48/92 -> concatenate/6108
  t48/93 -> concatenate/6109
  t48/94 -> concatenate/6110
  t48/95 -> concatenate/6111
  t48/96 -> concatenate/6112
  t48/97 -> concatenate/6113
  t48/98 -> concatenate/6114
  t48/99 -> concatenate/6115
  t48/100 -> concatenate/6116
  t48/101 -> concatenate/6117
  t48/102 -> concatenate/6118
  t48/103 -> concatenate/6119
  t48/104 -> concatenate/6120
  t48/105 -> concatenate/6121
  t48/106 -> concatenate/6122
  t48/107 -> concatenate/6123
  t48/108 -> concatenate/6124
  t48/109 -> concatenate/6125
  t48/110 -> concatenate/6126
  t48/111 -> concatenate/6127
  t48/112 -> concatenate/6128
  t48/113 -> concatenate/6129
  t48/114 -> concatenate/6130
  t48/115 -> concatenate/6131
  t48/116 -> concatenate/6132
  t48/117 -> concatenate/6133
  t48/118 -> concatenate/6134
  t48/119 -> concatenate/6135
  t48/120 -> concatenate/6136
  t48/121 -> concatenate/6137
  t48/122 -> concatenate/6138
  t48/123 -> concatenate/6139
  t48/124 -> concatenate/6140
  t48/125 -> concatenate/6141
  t48/126 -> concatenate/6142
  t48/127 -> concatenate/6143
  t48/128 -> concatenate/6144
  t49/1 -> concatenate/6145
  t49/2 -> concatenate/6146
  t49/3 -> concatenate/6147
  t49/4 -> concatenate/6148
  t49/5 -> concatenate/6149
  t49/6 -> concatenate/6150
  t49/7 -> concatenate/6151
  t49/8 -> concatenate/6152
  t49/9 -> concatenate/6153
  t49/10 -> concatenate/6154
  t49/11 -> concatenate/6155
  t49/12 -> concatenate/6156
  t49/13 -> concatenate/6157
  t49/14 -> concatenate/6158
  t49/15 -> concatenate/6159
  t49/16 -> concatenate/6160
  t49/17 -> concatenate/6161
  t49/18 -> concatenate/6162
  t49/19 -> concatenate/6163
  t49/20 -> concatenate/6164
  t49/21 -> concatenate/6165
  t49/22 -> concatenate/6166
  t49/23 -> concatenate/6167
  t49/24 -> concatenate/6168
  t49/25 -> concatenate/6169
  t49/26 -> concatenate/6170
  t49/27 -> concatenate/6171
  t49/28 -> concatenate/6172
  t49/29 -> concatenate/6173
  t49/30 -> concatenate/6174
  t49/31 -> concatenate/6175
  t49/32 -> concatenate/6176
  t49/33 -> concatenate/6177
  t49/34 -> concatenate/6178
  t49/35 -> concatenate/6179
  t49/36 -> concatenate/6180
  t49/37 -> concatenate/6181
  t49/38 -> concatenate/6182
  t49/39 -> concatenate/6183
  t49/40 -> concatenate/6184
  t49/41 -> concatenate/6185
  t49/42 -> concatenate/6186
  t49/43 -> concatenate/6187
  t49/44 -> concatenate/6188
  t49/45 -> concatenate/6189
  t49/46 -> concatenate/6190
  t49/47 -> concatenate/6191
  t49/48 -> concatenate/6192
  t49/49 -> concatenate/6193
  t49/50 -> concatenate/6194
  t49/51 -> concatenate/6195
  t49/52 -> concatenate/6196
  t49/53 -> concatenate/6197
  t49/54 -> concatenate/6198
  t49/55 -> concatenate/6199
  t49/56 -> concatenate/6200
  t49/57 -> concatenate/6201
  t49/58 -> concatenate/6202
  t49/59 -> concatenate/6203
  t49/60 -> concatenate/6204
  t49/61 -> concatenate/6205
  t49/62 -> concatenate/6206
  t49/63 -> concatenate/6207
  t49/64 -> concatenate/6208
  t49/65 -> concatenate/6209
  t49/66 -> concatenate/6210
  t49/67 -> concatenate/6211
  t49/68 -> concatenate/6212
  t49/69 -> concatenate/6213
  t49/70 -> concatenate/6214
  t49/71 -> concatenate/6215
  t49/72 -> concatenate/6216
  t49/73 -> concatenate/6217
  t49/74 -> concatenate/6218
  t49/75 -> concatenate/6219
  t49/76 -> concatenate/6220
  t49/77 -> concatenate/6221
  t49/78 -> concatenate/6222
  t49/79 -> concatenate/6223
  t49/80 -> concatenate/6224
  t49/81 -> concatenate/6225
  t49/82 -> concatenate/6226
  t49/83 -> concatenate/6227
  t49/84 -> concatenate/6228
  t49/85 -> concatenate/6229
  t49/86 -> concatenate/6230
  t49/87 -> concatenate/6231
  t49/88 -> concatenate/6232
  t49/89 -> concatenate/6233
  t49/90 -> concatenate/6234
  t49/91 -> concatenate/6235
  t49/92 -> concatenate/6236
  t49/93 -> concatenate/6237
  t49/94 -> concatenate/6238
  t49/95 -> concatenate/6239
  t49/96 -> concatenate/6240
  t49/97 -> concatenate/6241
  t49/98 -> concatenate/6242
  t49/99 -> concatenate/6243
  t49/100 -> concatenate/6244
  t49/101 -> concatenate/6245
  t49/102 -> concatenate/6246
  t49/103 -> concatenate/6247
  t49/104 -> concatenate/6248
  t49/105 -> concatenate/6249
  t49/106 -> concatenate/6250
  t49/107 -> concatenate/6251
  t49/108 -> concatenate/6252
  t49/109 -> concatenate/6253
  t49/110 -> concatenate/6254
  t49/111 -> concatenate/6255
  t49/112 -> concatenate/6256
  t49/113 -> concatenate/6257
  t49/114 -> concatenate/6258
  t49/115 -> concatenate/6259
  t49/116 -> concatenate/6260
  t49/117 -> concatenate/6261
  t49/118 -> concatenate/6262
  t49/119 -> concatenate/6263
  t49/120 -> concatenate/6264
  t49/121 -> concatenate/6265
  t49/122 -> concatenate/6266
  t49/123 -> concatenate/6267
  t49/124 -> concatenate/6268
  t49/125 -> concatenate/6269
  t49/126 -> concatenate/6270
  t49/127 -> concatenate/6271
  t49/128 -> concatenate/6272
  t50/1 -> concatenate/6273
  t50/2 -> concatenate/6274
  t50/3 -> concatenate/6275
  t50/4 -> concatenate/6276
  t50/5 -> concatenate/6277
  t50/6 -> concatenate/6278
  t50/7 -> concatenate/6279
  t50/8 -> concatenate/6280
  t50/9 -> concatenate/6281
  t50/10 -> concatenate/6282
  t50/11 -> concatenate/6283
  t50/12 -> concatenate/6284
  t50/13 -> concatenate/6285
  t50/14 -> concatenate/6286
  t50/15 -> concatenate/6287
  t50/16 -> concatenate/6288
  t50/17 -> concatenate/6289
  t50/18 -> concatenate/6290
  t50/19 -> concatenate/6291
  t50/20 -> concatenate/6292
  t50/21 -> concatenate/6293
  t50/22 -> concatenate/6294
  t50/23 -> concatenate/6295
  t50/24 -> concatenate/6296
  t50/25 -> concatenate/6297
  t50/26 -> concatenate/6298
  t50/27 -> concatenate/6299
  t50/28 -> concatenate/6300
  t50/29 -> concatenate/6301
  t50/30 -> concatenate/6302
  t50/31 -> concatenate/6303
  t50/32 -> concatenate/6304
  t50/33 -> concatenate/6305
  t50/34 -> concatenate/6306
  t50/35 -> concatenate/6307
  t50/36 -> concatenate/6308
  t50/37 -> concatenate/6309
  t50/38 -> concatenate/6310
  t50/39 -> concatenate/6311
  t50/40 -> concatenate/6312
  t50/41 -> concatenate/6313
  t50/42 -> concatenate/6314
  t50/43 -> concatenate/6315
  t50/44 -> concatenate/6316
  t50/45 -> concatenate/6317
  t50/46 -> concatenate/6318
  t50/47 -> concatenate/6319
  t50/48 -> concatenate/6320
  t50/49 -> concatenate/6321
  t50/50 -> concatenate/6322
  t50/51 -> concatenate/6323
  t50/52 -> concatenate/6324
  t50/53 -> concatenate/6325
  t50/54 -> concatenate/6326
  t50/55 -> concatenate/6327
  t50/56 -> concatenate/6328
  t50/57 -> concatenate/6329
  t50/58 -> concatenate/6330
  t50/59 -> concatenate/6331
  t50/60 -> concatenate/6332
  t50/61 -> concatenate/6333
  t50/62 -> concatenate/6334
  t50/63 -> concatenate/6335
  t50/64 -> concatenate/6336
  t50/65 -> concatenate/6337
  t50/66 -> concatenate/6338
  t50/67 -> concatenate/6339
  t50/68 -> concatenate/6340
  t50/69 -> concatenate/6341
  t50/70 -> concatenate/6342
  t50/71 -> concatenate/6343
  t50/72 -> concatenate/6344
  t50/73 -> concatenate/6345
  t50/74 -> concatenate/6346
  t50/75 -> concatenate/6347
  t50/76 -> concatenate/6348
  t50/77 -> concatenate/6349
  t50/78 -> concatenate/6350
  t50/79 -> concatenate/6351
  t50/80 -> concatenate/6352
  t50/81 -> concatenate/6353
  t50/82 -> concatenate/6354
  t50/83 -> concatenate/6355
  t50/84 -> concatenate/6356
  t50/85 -> concatenate/6357
  t50/86 -> concatenate/6358
  t50/87 -> concatenate/6359
  t50/88 -> concatenate/6360
  t50/89 -> concatenate/6361
  t50/90 -> concatenate/6362
  t50/91 -> concatenate/6363
  t50/92 -> concatenate/6364
  t50/93 -> concatenate/6365
  t50/94 -> concatenate/6366
  t50/95 -> concatenate/6367
  t50/96 -> concatenate/6368
  t50/97 -> concatenate/6369
  t50/98 -> concatenate/6370
  t50/99 -> concatenate/6371
  t50/100 -> concatenate/6372
  t50/101 -> concatenate/6373
  t50/102 -> concatenate/6374
  t50/103 -> concatenate/6375
  t50/104 -> concatenate/6376
  t50/105 -> concatenate/6377
  t50/106 -> concatenate/6378
  t50/107 -> concatenate/6379
  t50/108 -> concatenate/6380
  t50/109 -> concatenate/6381
  t50/110 -> concatenate/6382
  t50/111 -> concatenate/6383
  t50/112 -> concatenate/6384
  t50/113 -> concatenate/6385
  t50/114 -> concatenate/6386
  t50/115 -> concatenate/6387
  t50/116 -> concatenate/6388
  t50/117 -> concatenate/6389
  t50/118 -> concatenate/6390
  t50/119 -> concatenate/6391
  t50/120 -> concatenate/6392
  t50/121 -> concatenate/6393
  t50/122 -> concatenate/6394
  t50/123 -> concatenate/6395
  t50/124 -> concatenate/6396
  t50/125 -> concatenate/6397
  t50/126 -> concatenate/6398
  t50/127 -> concatenate/6399
  t50/128 -> concatenate/6400
  t51/1 -> concatenate/6401
  t51/2 -> concatenate/6402
  t51/3 -> concatenate/6403
  t51/4 -> concatenate/6404
  t51/5 -> concatenate/6405
  t51/6 -> concatenate/6406
  t51/7 -> concatenate/6407
  t51/8 -> concatenate/6408
  t51/9 -> concatenate/6409
  t51/10 -> concatenate/6410
  t51/11 -> concatenate/6411
  t51/12 -> concatenate/6412
  t51/13 -> concatenate/6413
  t51/14 -> concatenate/6414
  t51/15 -> concatenate/6415
  t51/16 -> concatenate/6416
  t51/17 -> concatenate/6417
  t51/18 -> concatenate/6418
  t51/19 -> concatenate/6419
  t51/20 -> concatenate/6420
  t51/21 -> concatenate/6421
  t51/22 -> concatenate/6422
  t51/23 -> concatenate/6423
  t51/24 -> concatenate/6424
  t51/25 -> concatenate/6425
  t51/26 -> concatenate/6426
  t51/27 -> concatenate/6427
  t51/28 -> concatenate/6428
  t51/29 -> concatenate/6429
  t51/30 -> concatenate/6430
  t51/31 -> concatenate/6431
  t51/32 -> concatenate/6432
  t51/33 -> concatenate/6433
  t51/34 -> concatenate/6434
  t51/35 -> concatenate/6435
  t51/36 -> concatenate/6436
  t51/37 -> concatenate/6437
  t51/38 -> concatenate/6438
  t51/39 -> concatenate/6439
  t51/40 -> concatenate/6440
  t51/41 -> concatenate/6441
  t51/42 -> concatenate/6442
  t51/43 -> concatenate/6443
  t51/44 -> concatenate/6444
  t51/45 -> concatenate/6445
  t51/46 -> concatenate/6446
  t51/47 -> concatenate/6447
  t51/48 -> concatenate/6448
  t51/49 -> concatenate/6449
  t51/50 -> concatenate/6450
  t51/51 -> concatenate/6451
  t51/52 -> concatenate/6452
  t51/53 -> concatenate/6453
  t51/54 -> concatenate/6454
  t51/55 -> concatenate/6455
  t51/56 -> concatenate/6456
  t51/57 -> concatenate/6457
  t51/58 -> concatenate/6458
  t51/59 -> concatenate/6459
  t51/60 -> concatenate/6460
  t51/61 -> concatenate/6461
  t51/62 -> concatenate/6462
  t51/63 -> concatenate/6463
  t51/64 -> concatenate/6464
  t51/65 -> concatenate/6465
  t51/66 -> concatenate/6466
  t51/67 -> concatenate/6467
  t51/68 -> concatenate/6468
  t51/69 -> concatenate/6469
  t51/70 -> concatenate/6470
  t51/71 -> concatenate/6471
  t51/72 -> concatenate/6472
  t51/73 -> concatenate/6473
  t51/74 -> concatenate/6474
  t51/75 -> concatenate/6475
  t51/76 -> concatenate/6476
  t51/77 -> concatenate/6477
  t51/78 -> concatenate/6478
  t51/79 -> concatenate/6479
  t51/80 -> concatenate/6480
  t51/81 -> concatenate/6481
  t51/82 -> concatenate/6482
  t51/83 -> concatenate/6483
  t51/84 -> concatenate/6484
  t51/85 -> concatenate/6485
  t51/86 -> concatenate/6486
  t51/87 -> concatenate/6487
  t51/88 -> concatenate/6488
  t51/89 -> concatenate/6489
  t51/90 -> concatenate/6490
  t51/91 -> concatenate/6491
  t51/92 -> concatenate/6492
  t51/93 -> concatenate/6493
  t51/94 -> concatenate/6494
  t51/95 -> concatenate/6495
  t51/96 -> concatenate/6496
  t51/97 -> concatenate/6497
  t51/98 -> concatenate/6498
  t51/99 -> concatenate/6499
  t51/100 -> concatenate/6500
  t51/101 -> concatenate/6501
  t51/102 -> concatenate/6502
  t51/103 -> concatenate/6503
  t51/104 -> concatenate/6504
  t51/105 -> concatenate/6505
  t51/106 -> concatenate/6506
  t51/107 -> concatenate/6507
  t51/108 -> concatenate/6508
  t51/109 -> concatenate/6509
  t51/110 -> concatenate/6510
  t51/111 -> concatenate/6511
  t51/112 -> concatenate/6512
  t51/113 -> concatenate/6513
  t51/114 -> concatenate/6514
  t51/115 -> concatenate/6515
  t51/116 -> concatenate/6516
  t51/117 -> concatenate/6517
  t51/118 -> concatenate/6518
  t51/119 -> concatenate/6519
  t51/120 -> concatenate/6520
  t51/121 -> concatenate/6521
  t51/122 -> concatenate/6522
  t51/123 -> concatenate/6523
  t51/124 -> concatenate/6524
  t51/125 -> concatenate/6525
  t51/126 -> concatenate/6526
  t51/127 -> concatenate/6527
  t51/128 -> concatenate/6528
  t52/1 -> concatenate/6529
  t52/2 -> concatenate/6530
  t52/3 -> concatenate/6531
  t52/4 -> concatenate/6532
  t52/5 -> concatenate/6533
  t52/6 -> concatenate/6534
  t52/7 -> concatenate/6535
  t52/8 -> concatenate/6536
  t52/9 -> concatenate/6537
  t52/10 -> concatenate/6538
  t52/11 -> concatenate/6539
  t52/12 -> concatenate/6540
  t52/13 -> concatenate/6541
  t52/14 -> concatenate/6542
  t52/15 -> concatenate/6543
  t52/16 -> concatenate/6544
  t52/17 -> concatenate/6545
  t52/18 -> concatenate/6546
  t52/19 -> concatenate/6547
  t52/20 -> concatenate/6548
  t52/21 -> concatenate/6549
  t52/22 -> concatenate/6550
  t52/23 -> concatenate/6551
  t52/24 -> concatenate/6552
  t52/25 -> concatenate/6553
  t52/26 -> concatenate/6554
  t52/27 -> concatenate/6555
  t52/28 -> concatenate/6556
  t52/29 -> concatenate/6557
  t52/30 -> concatenate/6558
  t52/31 -> concatenate/6559
  t52/32 -> concatenate/6560
  t52/33 -> concatenate/6561
  t52/34 -> concatenate/6562
  t52/35 -> concatenate/6563
  t52/36 -> concatenate/6564
  t52/37 -> concatenate/6565
  t52/38 -> concatenate/6566
  t52/39 -> concatenate/6567
  t52/40 -> concatenate/6568
  t52/41 -> concatenate/6569
  t52/42 -> concatenate/6570
  t52/43 -> concatenate/6571
  t52/44 -> concatenate/6572
  t52/45 -> concatenate/6573
  t52/46 -> concatenate/6574
  t52/47 -> concatenate/6575
  t52/48 -> concatenate/6576
  t52/49 -> concatenate/6577
  t52/50 -> concatenate/6578
  t52/51 -> concatenate/6579
  t52/52 -> concatenate/6580
  t52/53 -> concatenate/6581
  t52/54 -> concatenate/6582
  t52/55 -> concatenate/6583
  t52/56 -> concatenate/6584
  t52/57 -> concatenate/6585
  t52/58 -> concatenate/6586
  t52/59 -> concatenate/6587
  t52/60 -> concatenate/6588
  t52/61 -> concatenate/6589
  t52/62 -> concatenate/6590
  t52/63 -> concatenate/6591
  t52/64 -> concatenate/6592
  t52/65 -> concatenate/6593
  t52/66 -> concatenate/6594
  t52/67 -> concatenate/6595
  t52/68 -> concatenate/6596
  t52/69 -> concatenate/6597
  t52/70 -> concatenate/6598
  t52/71 -> concatenate/6599
  t52/72 -> concatenate/6600
  t52/73 -> concatenate/6601
  t52/74 -> concatenate/6602
  t52/75 -> concatenate/6603
  t52/76 -> concatenate/6604
  t52/77 -> concatenate/6605
  t52/78 -> concatenate/6606
  t52/79 -> concatenate/6607
  t52/80 -> concatenate/6608
  t52/81 -> concatenate/6609
  t52/82 -> concatenate/6610
  t52/83 -> concatenate/6611
  t52/84 -> concatenate/6612
  t52/85 -> concatenate/6613
  t52/86 -> concatenate/6614
  t52/87 -> concatenate/6615
  t52/88 -> concatenate/6616
  t52/89 -> concatenate/6617
  t52/90 -> concatenate/6618
  t52/91 -> concatenate/6619
  t52/92 -> concatenate/6620
  t52/93 -> concatenate/6621
  t52/94 -> concatenate/6622
  t52/95 -> concatenate/6623
  t52/96 -> concatenate/6624
  t52/97 -> concatenate/6625
  t52/98 -> concatenate/6626
  t52/99 -> concatenate/6627
  t52/100 -> concatenate/6628
  t52/101 -> concatenate/6629
  t52/102 -> concatenate/6630
  t52/103 -> concatenate/6631
  t52/104 -> concatenate/6632
  t52/105 -> concatenate/6633
  t52/106 -> concatenate/6634
  t52/107 -> concatenate/6635
  t52/108 -> concatenate/6636
  t52/109 -> concatenate/6637
  t52/110 -> concatenate/6638
  t52/111 -> concatenate/6639
  t52/112 -> concatenate/6640
  t52/113 -> concatenate/6641
  t52/114 -> concatenate/6642
  t52/115 -> concatenate/6643
  t52/116 -> concatenate/6644
  t52/117 -> concatenate/6645
  t52/118 -> concatenate/6646
  t52/119 -> concatenate/6647
  t52/120 -> concatenate/6648
  t52/121 -> concatenate/6649
  t52/122 -> concatenate/6650
  t52/123 -> concatenate/6651
  t52/124 -> concatenate/6652
  t52/125 -> concatenate/6653
  t52/126 -> concatenate/6654
  t52/127 -> concatenate/6655
  t52/128 -> concatenate/6656
  t53/1 -> concatenate/6657
  t53/2 -> concatenate/6658
  t53/3 -> concatenate/6659
  t53/4 -> concatenate/6660
  t53/5 -> concatenate/6661
  t53/6 -> concatenate/6662
  t53/7 -> concatenate/6663
  t53/8 -> concatenate/6664
  t53/9 -> concatenate/6665
  t53/10 -> concatenate/6666
  t53/11 -> concatenate/6667
  t53/12 -> concatenate/6668
  t53/13 -> concatenate/6669
  t53/14 -> concatenate/6670
  t53/15 -> concatenate/6671
  t53/16 -> concatenate/6672
  t53/17 -> concatenate/6673
  t53/18 -> concatenate/6674
  t53/19 -> concatenate/6675
  t53/20 -> concatenate/6676
  t53/21 -> concatenate/6677
  t53/22 -> concatenate/6678
  t53/23 -> concatenate/6679
  t53/24 -> concatenate/6680
  t53/25 -> concatenate/6681
  t53/26 -> concatenate/6682
  t53/27 -> concatenate/6683
  t53/28 -> concatenate/6684
  t53/29 -> concatenate/6685
  t53/30 -> concatenate/6686
  t53/31 -> concatenate/6687
  t53/32 -> concatenate/6688
  t53/33 -> concatenate/6689
  t53/34 -> concatenate/6690
  t53/35 -> concatenate/6691
  t53/36 -> concatenate/6692
  t53/37 -> concatenate/6693
  t53/38 -> concatenate/6694
  t53/39 -> concatenate/6695
  t53/40 -> concatenate/6696
  t53/41 -> concatenate/6697
  t53/42 -> concatenate/6698
  t53/43 -> concatenate/6699
  t53/44 -> concatenate/6700
  t53/45 -> concatenate/6701
  t53/46 -> concatenate/6702
  t53/47 -> concatenate/6703
  t53/48 -> concatenate/6704
  t53/49 -> concatenate/6705
  t53/50 -> concatenate/6706
  t53/51 -> concatenate/6707
  t53/52 -> concatenate/6708
  t53/53 -> concatenate/6709
  t53/54 -> concatenate/6710
  t53/55 -> concatenate/6711
  t53/56 -> concatenate/6712
  t53/57 -> concatenate/6713
  t53/58 -> concatenate/6714
  t53/59 -> concatenate/6715
  t53/60 -> concatenate/6716
  t53/61 -> concatenate/6717
  t53/62 -> concatenate/6718
  t53/63 -> concatenate/6719
  t53/64 -> concatenate/6720
  t53/65 -> concatenate/6721
  t53/66 -> concatenate/6722
  t53/67 -> concatenate/6723
  t53/68 -> concatenate/6724
  t53/69 -> concatenate/6725
  t53/70 -> concatenate/6726
  t53/71 -> concatenate/6727
  t53/72 -> concatenate/6728
  t53/73 -> concatenate/6729
  t53/74 -> concatenate/6730
  t53/75 -> concatenate/6731
  t53/76 -> concatenate/6732
  t53/77 -> concatenate/6733
  t53/78 -> concatenate/6734
  t53/79 -> concatenate/6735
  t53/80 -> concatenate/6736
  t53/81 -> concatenate/6737
  t53/82 -> concatenate/6738
  t53/83 -> concatenate/6739
  t53/84 -> concatenate/6740
  t53/85 -> concatenate/6741
  t53/86 -> concatenate/6742
  t53/87 -> concatenate/6743
  t53/88 -> concatenate/6744
  t53/89 -> concatenate/6745
  t53/90 -> concatenate/6746
  t53/91 -> concatenate/6747
  t53/92 -> concatenate/6748
  t53/93 -> concatenate/6749
  t53/94 -> concatenate/6750
  t53/95 -> concatenate/6751
  t53/96 -> concatenate/6752
  t53/97 -> concatenate/6753
  t53/98 -> concatenate/6754
  t53/99 -> concatenate/6755
  t53/100 -> concatenate/6756
  t53/101 -> concatenate/6757
  t53/102 -> concatenate/6758
  t53/103 -> concatenate/6759
  t53/104 -> concatenate/6760
  t53/105 -> concatenate/6761
  t53/106 -> concatenate/6762
  t53/107 -> concatenate/6763
  t53/108 -> concatenate/6764
  t53/109 -> concatenate/6765
  t53/110 -> concatenate/6766
  t53/111 -> concatenate/6767
  t53/112 -> concatenate/6768
  t53/113 -> concatenate/6769
  t53/114 -> concatenate/6770
  t53/115 -> concatenate/6771
  t53/116 -> concatenate/6772
  t53/117 -> concatenate/6773
  t53/118 -> concatenate/6774
  t53/119 -> concatenate/6775
  t53/120 -> concatenate/6776
  t53/121 -> concatenate/6777
  t53/122 -> concatenate/6778
  t53/123 -> concatenate/6779
  t53/124 -> concatenate/6780
  t53/125 -> concatenate/6781
  t53/126 -> concatenate/6782
  t53/127 -> concatenate/6783
  t53/128 -> concatenate/6784
  t54/1 -> concatenate/6785
  t54/2 -> concatenate/6786
  t54/3 -> concatenate/6787
  t54/4 -> concatenate/6788
  t54/5 -> concatenate/6789
  t54/6 -> concatenate/6790
  t54/7 -> concatenate/6791
  t54/8 -> concatenate/6792
  t54/9 -> concatenate/6793
  t54/10 -> concatenate/6794
  t54/11 -> concatenate/6795
  t54/12 -> concatenate/6796
  t54/13 -> concatenate/6797
  t54/14 -> concatenate/6798
  t54/15 -> concatenate/6799
  t54/16 -> concatenate/6800
  t54/17 -> concatenate/6801
  t54/18 -> concatenate/6802
  t54/19 -> concatenate/6803
  t54/20 -> concatenate/6804
  t54/21 -> concatenate/6805
  t54/22 -> concatenate/6806
  t54/23 -> concatenate/6807
  t54/24 -> concatenate/6808
  t54/25 -> concatenate/6809
  t54/26 -> concatenate/6810
  t54/27 -> concatenate/6811
  t54/28 -> concatenate/6812
  t54/29 -> concatenate/6813
  t54/30 -> concatenate/6814
  t54/31 -> concatenate/6815
  t54/32 -> concatenate/6816
  t54/33 -> concatenate/6817
  t54/34 -> concatenate/6818
  t54/35 -> concatenate/6819
  t54/36 -> concatenate/6820
  t54/37 -> concatenate/6821
  t54/38 -> concatenate/6822
  t54/39 -> concatenate/6823
  t54/40 -> concatenate/6824
  t54/41 -> concatenate/6825
  t54/42 -> concatenate/6826
  t54/43 -> concatenate/6827
  t54/44 -> concatenate/6828
  t54/45 -> concatenate/6829
  t54/46 -> concatenate/6830
  t54/47 -> concatenate/6831
  t54/48 -> concatenate/6832
  t54/49 -> concatenate/6833
  t54/50 -> concatenate/6834
  t54/51 -> concatenate/6835
  t54/52 -> concatenate/6836
  t54/53 -> concatenate/6837
  t54/54 -> concatenate/6838
  t54/55 -> concatenate/6839
  t54/56 -> concatenate/6840
  t54/57 -> concatenate/6841
  t54/58 -> concatenate/6842
  t54/59 -> concatenate/6843
  t54/60 -> concatenate/6844
  t54/61 -> concatenate/6845
  t54/62 -> concatenate/6846
  t54/63 -> concatenate/6847
  t54/64 -> concatenate/6848
  t54/65 -> concatenate/6849
  t54/66 -> concatenate/6850
  t54/67 -> concatenate/6851
  t54/68 -> concatenate/6852
  t54/69 -> concatenate/6853
  t54/70 -> concatenate/6854
  t54/71 -> concatenate/6855
  t54/72 -> concatenate/6856
  t54/73 -> concatenate/6857
  t54/74 -> concatenate/6858
  t54/75 -> concatenate/6859
  t54/76 -> concatenate/6860
  t54/77 -> concatenate/6861
  t54/78 -> concatenate/6862
  t54/79 -> concatenate/6863
  t54/80 -> concatenate/6864
  t54/81 -> concatenate/6865
  t54/82 -> concatenate/6866
  t54/83 -> concatenate/6867
  t54/84 -> concatenate/6868
  t54/85 -> concatenate/6869
  t54/86 -> concatenate/6870
  t54/87 -> concatenate/6871
  t54/88 -> concatenate/6872
  t54/89 -> concatenate/6873
  t54/90 -> concatenate/6874
  t54/91 -> concatenate/6875
  t54/92 -> concatenate/6876
  t54/93 -> concatenate/6877
  t54/94 -> concatenate/6878
  t54/95 -> concatenate/6879
  t54/96 -> concatenate/6880
  t54/97 -> concatenate/6881
  t54/98 -> concatenate/6882
  t54/99 -> concatenate/6883
  t54/100 -> concatenate/6884
  t54/101 -> concatenate/6885
  t54/102 -> concatenate/6886
  t54/103 -> concatenate/6887
  t54/104 -> concatenate/6888
  t54/105 -> concatenate/6889
  t54/106 -> concatenate/6890
  t54/107 -> concatenate/6891
  t54/108 -> concatenate/6892
  t54/109 -> concatenate/6893
  t54/110 -> concatenate/6894
  t54/111 -> concatenate/6895
  t54/112 -> concatenate/6896
  t54/113 -> concatenate/6897
  t54/114 -> concatenate/6898
  t54/115 -> concatenate/6899
  t54/116 -> concatenate/6900
  t54/117 -> concatenate/6901
  t54/118 -> concatenate/6902
  t54/119 -> concatenate/6903
  t54/120 -> concatenate/6904
  t54/121 -> concatenate/6905
  t54/122 -> concatenate/6906
  t54/123 -> concatenate/6907
  t54/124 -> concatenate/6908
  t54/125 -> concatenate/6909
  t54/126 -> concatenate/6910
  t54/127 -> concatenate/6911
  t54/128 -> concatenate/6912
  t55/1 -> concatenate/6913
  t55/2 -> concatenate/6914
  t55/3 -> concatenate/6915
  t55/4 -> concatenate/6916
  t55/5 -> concatenate/6917
  t55/6 -> concatenate/6918
  t55/7 -> concatenate/6919
  t55/8 -> concatenate/6920
  t55/9 -> concatenate/6921
  t55/10 -> concatenate/6922
  t55/11 -> concatenate/6923
  t55/12 -> concatenate/6924
  t55/13 -> concatenate/6925
  t55/14 -> concatenate/6926
  t55/15 -> concatenate/6927
  t55/16 -> concatenate/6928
  t55/17 -> concatenate/6929
  t55/18 -> concatenate/6930
  t55/19 -> concatenate/6931
  t55/20 -> concatenate/6932
  t55/21 -> concatenate/6933
  t55/22 -> concatenate/6934
  t55/23 -> concatenate/6935
  t55/24 -> concatenate/6936
  t55/25 -> concatenate/6937
  t55/26 -> concatenate/6938
  t55/27 -> concatenate/6939
  t55/28 -> concatenate/6940
  t55/29 -> concatenate/6941
  t55/30 -> concatenate/6942
  t55/31 -> concatenate/6943
  t55/32 -> concatenate/6944
  t55/33 -> concatenate/6945
  t55/34 -> concatenate/6946
  t55/35 -> concatenate/6947
  t55/36 -> concatenate/6948
  t55/37 -> concatenate/6949
  t55/38 -> concatenate/6950
  t55/39 -> concatenate/6951
  t55/40 -> concatenate/6952
  t55/41 -> concatenate/6953
  t55/42 -> concatenate/6954
  t55/43 -> concatenate/6955
  t55/44 -> concatenate/6956
  t55/45 -> concatenate/6957
  t55/46 -> concatenate/6958
  t55/47 -> concatenate/6959
  t55/48 -> concatenate/6960
  t55/49 -> concatenate/6961
  t55/50 -> concatenate/6962
  t55/51 -> concatenate/6963
  t55/52 -> concatenate/6964
  t55/53 -> concatenate/6965
  t55/54 -> concatenate/6966
  t55/55 -> concatenate/6967
  t55/56 -> concatenate/6968
  t55/57 -> concatenate/6969
  t55/58 -> concatenate/6970
  t55/59 -> concatenate/6971
  t55/60 -> concatenate/6972
  t55/61 -> concatenate/6973
  t55/62 -> concatenate/6974
  t55/63 -> concatenate/6975
  t55/64 -> concatenate/6976
  t55/65 -> concatenate/6977
  t55/66 -> concatenate/6978
  t55/67 -> concatenate/6979
  t55/68 -> concatenate/6980
  t55/69 -> concatenate/6981
  t55/70 -> concatenate/6982
  t55/71 -> concatenate/6983
  t55/72 -> concatenate/6984
  t55/73 -> concatenate/6985
  t55/74 -> concatenate/6986
  t55/75 -> concatenate/6987
  t55/76 -> concatenate/6988
  t55/77 -> concatenate/6989
  t55/78 -> concatenate/6990
  t55/79 -> concatenate/6991
  t55/80 -> concatenate/6992
  t55/81 -> concatenate/6993
  t55/82 -> concatenate/6994
  t55/83 -> concatenate/6995
  t55/84 -> concatenate/6996
  t55/85 -> concatenate/6997
  t55/86 -> concatenate/6998
  t55/87 -> concatenate/6999
  t55/88 -> concatenate/7000
  t55/89 -> concatenate/7001
  t55/90 -> concatenate/7002
  t55/91 -> concatenate/7003
  t55/92 -> concatenate/7004
  t55/93 -> concatenate/7005
  t55/94 -> concatenate/7006
  t55/95 -> concatenate/7007
  t55/96 -> concatenate/7008
  t55/97 -> concatenate/7009
  t55/98 -> concatenate/7010
  t55/99 -> concatenate/7011
  t55/100 -> concatenate/7012
  t55/101 -> concatenate/7013
  t55/102 -> concatenate/7014
  t55/103 -> concatenate/7015
  t55/104 -> concatenate/7016
  t55/105 -> concatenate/7017
  t55/106 -> concatenate/7018
  t55/107 -> concatenate/7019
  t55/108 -> concatenate/7020
  t55/109 -> concatenate/7021
  t55/110 -> concatenate/7022
  t55/111 -> concatenate/7023
  t55/112 -> concatenate/7024
  t55/113 -> concatenate/7025
  t55/114 -> concatenate/7026
  t55/115 -> concatenate/7027
  t55/116 -> concatenate/7028
  t55/117 -> concatenate/7029
  t55/118 -> concatenate/7030
  t55/119 -> concatenate/7031
  t55/120 -> concatenate/7032
  t55/121 -> concatenate/7033
  t55/122 -> concatenate/7034
  t55/123 -> concatenate/7035
  t55/124 -> concatenate/7036
  t55/125 -> concatenate/7037
  t55/126 -> concatenate/7038
  t55/127 -> concatenate/7039
  t55/128 -> concatenate/7040
  t56/1 -> concatenate/7041
  t56/2 -> concatenate/7042
  t56/3 -> concatenate/7043
  t56/4 -> concatenate/7044
  t56/5 -> concatenate/7045
  t56/6 -> concatenate/7046
  t56/7 -> concatenate/7047
  t56/8 -> concatenate/7048
  t56/9 -> concatenate/7049
  t56/10 -> concatenate/7050
  t56/11 -> concatenate/7051
  t56/12 -> concatenate/7052
  t56/13 -> concatenate/7053
  t56/14 -> concatenate/7054
  t56/15 -> concatenate/7055
  t56/16 -> concatenate/7056
  t56/17 -> concatenate/7057
  t56/18 -> concatenate/7058
  t56/19 -> concatenate/7059
  t56/20 -> concatenate/7060
  t56/21 -> concatenate/7061
  t56/22 -> concatenate/7062
  t56/23 -> concatenate/7063
  t56/24 -> concatenate/7064
  t56/25 -> concatenate/7065
  t56/26 -> concatenate/7066
  t56/27 -> concatenate/7067
  t56/28 -> concatenate/7068
  t56/29 -> concatenate/7069
  t56/30 -> concatenate/7070
  t56/31 -> concatenate/7071
  t56/32 -> concatenate/7072
  t56/33 -> concatenate/7073
  t56/34 -> concatenate/7074
  t56/35 -> concatenate/7075
  t56/36 -> concatenate/7076
  t56/37 -> concatenate/7077
  t56/38 -> concatenate/7078
  t56/39 -> concatenate/7079
  t56/40 -> concatenate/7080
  t56/41 -> concatenate/7081
  t56/42 -> concatenate/7082
  t56/43 -> concatenate/7083
  t56/44 -> concatenate/7084
  t56/45 -> concatenate/7085
  t56/46 -> concatenate/7086
  t56/47 -> concatenate/7087
  t56/48 -> concatenate/7088
  t56/49 -> concatenate/7089
  t56/50 -> concatenate/7090
  t56/51 -> concatenate/7091
  t56/52 -> concatenate/7092
  t56/53 -> concatenate/7093
  t56/54 -> concatenate/7094
  t56/55 -> concatenate/7095
  t56/56 -> concatenate/7096
  t56/57 -> concatenate/7097
  t56/58 -> concatenate/7098
  t56/59 -> concatenate/7099
  t56/60 -> concatenate/7100
  t56/61 -> concatenate/7101
  t56/62 -> concatenate/7102
  t56/63 -> concatenate/7103
  t56/64 -> concatenate/7104
  t56/65 -> concatenate/7105
  t56/66 -> concatenate/7106
  t56/67 -> concatenate/7107
  t56/68 -> concatenate/7108
  t56/69 -> concatenate/7109
  t56/70 -> concatenate/7110
  t56/71 -> concatenate/7111
  t56/72 -> concatenate/7112
  t56/73 -> concatenate/7113
  t56/74 -> concatenate/7114
  t56/75 -> concatenate/7115
  t56/76 -> concatenate/7116
  t56/77 -> concatenate/7117
  t56/78 -> concatenate/7118
  t56/79 -> concatenate/7119
  t56/80 -> concatenate/7120
  t56/81 -> concatenate/7121
  t56/82 -> concatenate/7122
  t56/83 -> concatenate/7123
  t56/84 -> concatenate/7124
  t56/85 -> concatenate/7125
  t56/86 -> concatenate/7126
  t56/87 -> concatenate/7127
  t56/88 -> concatenate/7128
  t56/89 -> concatenate/7129
  t56/90 -> concatenate/7130
  t56/91 -> concatenate/7131
  t56/92 -> concatenate/7132
  t56/93 -> concatenate/7133
  t56/94 -> concatenate/7134
  t56/95 -> concatenate/7135
  t56/96 -> concatenate/7136
  t56/97 -> concatenate/7137
  t56/98 -> concatenate/7138
  t56/99 -> concatenate/7139
  t56/100 -> concatenate/7140
  t56/101 -> concatenate/7141
  t56/102 -> concatenate/7142
  t56/103 -> concatenate/7143
  t56/104 -> concatenate/7144
  t56/105 -> concatenate/7145
  t56/106 -> concatenate/7146
  t56/107 -> concatenate/7147
  t56/108 -> concatenate/7148
  t56/109 -> concatenate/7149
  t56/110 -> concatenate/7150
  t56/111 -> concatenate/7151
  t56/112 -> concatenate/7152
  t56/113 -> concatenate/7153
  t56/114 -> concatenate/7154
  t56/115 -> concatenate/7155
  t56/116 -> concatenate/7156
  t56/117 -> concatenate/7157
  t56/118 -> concatenate/7158
  t56/119 -> concatenate/7159
  t56/120 -> concatenate/7160
  t56/121 -> concatenate/7161
  t56/122 -> concatenate/7162
  t56/123 -> concatenate/7163
  t56/124 -> concatenate/7164
  t56/125 -> concatenate/7165
  t56/126 -> concatenate/7166
  t56/127 -> concatenate/7167
  t56/128 -> concatenate/7168
  t57/1 -> concatenate/7169
  t57/2 -> concatenate/7170
  t57/3 -> concatenate/7171
  t57/4 -> concatenate/7172
  t57/5 -> concatenate/7173
  t57/6 -> concatenate/7174
  t57/7 -> concatenate/7175
  t57/8 -> concatenate/7176
  t57/9 -> concatenate/7177
  t57/10 -> concatenate/7178
  t57/11 -> concatenate/7179
  t57/12 -> concatenate/7180
  t57/13 -> concatenate/7181
  t57/14 -> concatenate/7182
  t57/15 -> concatenate/7183
  t57/16 -> concatenate/7184
  t57/17 -> concatenate/7185
  t57/18 -> concatenate/7186
  t57/19 -> concatenate/7187
  t57/20 -> concatenate/7188
  t57/21 -> concatenate/7189
  t57/22 -> concatenate/7190
  t57/23 -> concatenate/7191
  t57/24 -> concatenate/7192
  t57/25 -> concatenate/7193
  t57/26 -> concatenate/7194
  t57/27 -> concatenate/7195
  t57/28 -> concatenate/7196
  t57/29 -> concatenate/7197
  t57/30 -> concatenate/7198
  t57/31 -> concatenate/7199
  t57/32 -> concatenate/7200
  t57/33 -> concatenate/7201
  t57/34 -> concatenate/7202
  t57/35 -> concatenate/7203
  t57/36 -> concatenate/7204
  t57/37 -> concatenate/7205
  t57/38 -> concatenate/7206
  t57/39 -> concatenate/7207
  t57/40 -> concatenate/7208
  t57/41 -> concatenate/7209
  t57/42 -> concatenate/7210
  t57/43 -> concatenate/7211
  t57/44 -> concatenate/7212
  t57/45 -> concatenate/7213
  t57/46 -> concatenate/7214
  t57/47 -> concatenate/7215
  t57/48 -> concatenate/7216
  t57/49 -> concatenate/7217
  t57/50 -> concatenate/7218
  t57/51 -> concatenate/7219
  t57/52 -> concatenate/7220
  t57/53 -> concatenate/7221
  t57/54 -> concatenate/7222
  t57/55 -> concatenate/7223
  t57/56 -> concatenate/7224
  t57/57 -> concatenate/7225
  t57/58 -> concatenate/7226
  t57/59 -> concatenate/7227
  t57/60 -> concatenate/7228
  t57/61 -> concatenate/7229
  t57/62 -> concatenate/7230
  t57/63 -> concatenate/7231
  t57/64 -> concatenate/7232
  t57/65 -> concatenate/7233
  t57/66 -> concatenate/7234
  t57/67 -> concatenate/7235
  t57/68 -> concatenate/7236
  t57/69 -> concatenate/7237
  t57/70 -> concatenate/7238
  t57/71 -> concatenate/7239
  t57/72 -> concatenate/7240
  t57/73 -> concatenate/7241
  t57/74 -> concatenate/7242
  t57/75 -> concatenate/7243
  t57/76 -> concatenate/7244
  t57/77 -> concatenate/7245
  t57/78 -> concatenate/7246
  t57/79 -> concatenate/7247
  t57/80 -> concatenate/7248
  t57/81 -> concatenate/7249
  t57/82 -> concatenate/7250
  t57/83 -> concatenate/7251
  t57/84 -> concatenate/7252
  t57/85 -> concatenate/7253
  t57/86 -> concatenate/7254
  t57/87 -> concatenate/7255
  t57/88 -> concatenate/7256
  t57/89 -> concatenate/7257
  t57/90 -> concatenate/7258
  t57/91 -> concatenate/7259
  t57/92 -> concatenate/7260
  t57/93 -> concatenate/7261
  t57/94 -> concatenate/7262
  t57/95 -> concatenate/7263
  t57/96 -> concatenate/7264
  t57/97 -> concatenate/7265
  t57/98 -> concatenate/7266
  t57/99 -> concatenate/7267
  t57/100 -> concatenate/7268
  t57/101 -> concatenate/7269
  t57/102 -> concatenate/7270
  t57/103 -> concatenate/7271
  t57/104 -> concatenate/7272
  t57/105 -> concatenate/7273
  t57/106 -> concatenate/7274
  t57/107 -> concatenate/7275
  t57/108 -> concatenate/7276
  t57/109 -> concatenate/7277
  t57/110 -> concatenate/7278
  t57/111 -> concatenate/7279
  t57/112 -> concatenate/7280
  t57/113 -> concatenate/7281
  t57/114 -> concatenate/7282
  t57/115 -> concatenate/7283
  t57/116 -> concatenate/7284
  t57/117 -> concatenate/7285
  t57/118 -> concatenate/7286
  t57/119 -> concatenate/7287
  t57/120 -> concatenate/7288
  t57/121 -> concatenate/7289
  t57/122 -> concatenate/7290
  t57/123 -> concatenate/7291
  t57/124 -> concatenate/7292
  t57/125 -> concatenate/7293
  t57/126 -> concatenate/7294
  t57/127 -> concatenate/7295
  t57/128 -> concatenate/7296
  t58/1 -> concatenate/7297
  t58/2 -> concatenate/7298
  t58/3 -> concatenate/7299
  t58/4 -> concatenate/7300
  t58/5 -> concatenate/7301
  t58/6 -> concatenate/7302
  t58/7 -> concatenate/7303
  t58/8 -> concatenate/7304
  t58/9 -> concatenate/7305
  t58/10 -> concatenate/7306
  t58/11 -> concatenate/7307
  t58/12 -> concatenate/7308
  t58/13 -> concatenate/7309
  t58/14 -> concatenate/7310
  t58/15 -> concatenate/7311
  t58/16 -> concatenate/7312
  t58/17 -> concatenate/7313
  t58/18 -> concatenate/7314
  t58/19 -> concatenate/7315
  t58/20 -> concatenate/7316
  t58/21 -> concatenate/7317
  t58/22 -> concatenate/7318
  t58/23 -> concatenate/7319
  t58/24 -> concatenate/7320
  t58/25 -> concatenate/7321
  t58/26 -> concatenate/7322
  t58/27 -> concatenate/7323
  t58/28 -> concatenate/7324
  t58/29 -> concatenate/7325
  t58/30 -> concatenate/7326
  t58/31 -> concatenate/7327
  t58/32 -> concatenate/7328
  t58/33 -> concatenate/7329
  t58/34 -> concatenate/7330
  t58/35 -> concatenate/7331
  t58/36 -> concatenate/7332
  t58/37 -> concatenate/7333
  t58/38 -> concatenate/7334
  t58/39 -> concatenate/7335
  t58/40 -> concatenate/7336
  t58/41 -> concatenate/7337
  t58/42 -> concatenate/7338
  t58/43 -> concatenate/7339
  t58/44 -> concatenate/7340
  t58/45 -> concatenate/7341
  t58/46 -> concatenate/7342
  t58/47 -> concatenate/7343
  t58/48 -> concatenate/7344
  t58/49 -> concatenate/7345
  t58/50 -> concatenate/7346
  t58/51 -> concatenate/7347
  t58/52 -> concatenate/7348
  t58/53 -> concatenate/7349
  t58/54 -> concatenate/7350
  t58/55 -> concatenate/7351
  t58/56 -> concatenate/7352
  t58/57 -> concatenate/7353
  t58/58 -> concatenate/7354
  t58/59 -> concatenate/7355
  t58/60 -> concatenate/7356
  t58/61 -> concatenate/7357
  t58/62 -> concatenate/7358
  t58/63 -> concatenate/7359
  t58/64 -> concatenate/7360
  t58/65 -> concatenate/7361
  t58/66 -> concatenate/7362
  t58/67 -> concatenate/7363
  t58/68 -> concatenate/7364
  t58/69 -> concatenate/7365
  t58/70 -> concatenate/7366
  t58/71 -> concatenate/7367
  t58/72 -> concatenate/7368
  t58/73 -> concatenate/7369
  t58/74 -> concatenate/7370
  t58/75 -> concatenate/7371
  t58/76 -> concatenate/7372
  t58/77 -> concatenate/7373
  t58/78 -> concatenate/7374
  t58/79 -> concatenate/7375
  t58/80 -> concatenate/7376
  t58/81 -> concatenate/7377
  t58/82 -> concatenate/7378
  t58/83 -> concatenate/7379
  t58/84 -> concatenate/7380
  t58/85 -> concatenate/7381
  t58/86 -> concatenate/7382
  t58/87 -> concatenate/7383
  t58/88 -> concatenate/7384
  t58/89 -> concatenate/7385
  t58/90 -> concatenate/7386
  t58/91 -> concatenate/7387
  t58/92 -> concatenate/7388
  t58/93 -> concatenate/7389
  t58/94 -> concatenate/7390
  t58/95 -> concatenate/7391
  t58/96 -> concatenate/7392
  t58/97 -> concatenate/7393
  t58/98 -> concatenate/7394
  t58/99 -> concatenate/7395
  t58/100 -> concatenate/7396
  t58/101 -> concatenate/7397
  t58/102 -> concatenate/7398
  t58/103 -> concatenate/7399
  t58/104 -> concatenate/7400
  t58/105 -> concatenate/7401
  t58/106 -> concatenate/7402
  t58/107 -> concatenate/7403
  t58/108 -> concatenate/7404
  t58/109 -> concatenate/7405
  t58/110 -> concatenate/7406
  t58/111 -> concatenate/7407
  t58/112 -> concatenate/7408
  t58/113 -> concatenate/7409
  t58/114 -> concatenate/7410
  t58/115 -> concatenate/7411
  t58/116 -> concatenate/7412
  t58/117 -> concatenate/7413
  t58/118 -> concatenate/7414
  t58/119 -> concatenate/7415
  t58/120 -> concatenate/7416
  t58/121 -> concatenate/7417
  t58/122 -> concatenate/7418
  t58/123 -> concatenate/7419
  t58/124 -> concatenate/7420
  t58/125 -> concatenate/7421
  t58/126 -> concatenate/7422
  t58/127 -> concatenate/7423
  t58/128 -> concatenate/7424
  t59/1 -> concatenate/7425
  t59/2 -> concatenate/7426
  t59/3 -> concatenate/7427
  t59/4 -> concatenate/7428
  t59/5 -> concatenate/7429
  t59/6 -> concatenate/7430
  t59/7 -> concatenate/7431
  t59/8 -> concatenate/7432
  t59/9 -> concatenate/7433
  t59/10 -> concatenate/7434
  t59/11 -> concatenate/7435
  t59/12 -> concatenate/7436
  t59/13 -> concatenate/7437
  t59/14 -> concatenate/7438
  t59/15 -> concatenate/7439
  t59/16 -> concatenate/7440
  t59/17 -> concatenate/7441
  t59/18 -> concatenate/7442
  t59/19 -> concatenate/7443
  t59/20 -> concatenate/7444
  t59/21 -> concatenate/7445
  t59/22 -> concatenate/7446
  t59/23 -> concatenate/7447
  t59/24 -> concatenate/7448
  t59/25 -> concatenate/7449
  t59/26 -> concatenate/7450
  t59/27 -> concatenate/7451
  t59/28 -> concatenate/7452
  t59/29 -> concatenate/7453
  t59/30 -> concatenate/7454
  t59/31 -> concatenate/7455
  t59/32 -> concatenate/7456
  t59/33 -> concatenate/7457
  t59/34 -> concatenate/7458
  t59/35 -> concatenate/7459
  t59/36 -> concatenate/7460
  t59/37 -> concatenate/7461
  t59/38 -> concatenate/7462
  t59/39 -> concatenate/7463
  t59/40 -> concatenate/7464
  t59/41 -> concatenate/7465
  t59/42 -> concatenate/7466
  t59/43 -> concatenate/7467
  t59/44 -> concatenate/7468
  t59/45 -> concatenate/7469
  t59/46 -> concatenate/7470
  t59/47 -> concatenate/7471
  t59/48 -> concatenate/7472
  t59/49 -> concatenate/7473
  t59/50 -> concatenate/7474
  t59/51 -> concatenate/7475
  t59/52 -> concatenate/7476
  t59/53 -> concatenate/7477
  t59/54 -> concatenate/7478
  t59/55 -> concatenate/7479
  t59/56 -> concatenate/7480
  t59/57 -> concatenate/7481
  t59/58 -> concatenate/7482
  t59/59 -> concatenate/7483
  t59/60 -> concatenate/7484
  t59/61 -> concatenate/7485
  t59/62 -> concatenate/7486
  t59/63 -> concatenate/7487
  t59/64 -> concatenate/7488
  t59/65 -> concatenate/7489
  t59/66 -> concatenate/7490
  t59/67 -> concatenate/7491
  t59/68 -> concatenate/7492
  t59/69 -> concatenate/7493
  t59/70 -> concatenate/7494
  t59/71 -> concatenate/7495
  t59/72 -> concatenate/7496
  t59/73 -> concatenate/7497
  t59/74 -> concatenate/7498
  t59/75 -> concatenate/7499
  t59/76 -> concatenate/7500
  t59/77 -> concatenate/7501
  t59/78 -> concatenate/7502
  t59/79 -> concatenate/7503
  t59/80 -> concatenate/7504
  t59/81 -> concatenate/7505
  t59/82 -> concatenate/7506
  t59/83 -> concatenate/7507
  t59/84 -> concatenate/7508
  t59/85 -> concatenate/7509
  t59/86 -> concatenate/7510
  t59/87 -> concatenate/7511
  t59/88 -> concatenate/7512
  t59/89 -> concatenate/7513
  t59/90 -> concatenate/7514
  t59/91 -> concatenate/7515
  t59/92 -> concatenate/7516
  t59/93 -> concatenate/7517
  t59/94 -> concatenate/7518
  t59/95 -> concatenate/7519
  t59/96 -> concatenate/7520
  t59/97 -> concatenate/7521
  t59/98 -> concatenate/7522
  t59/99 -> concatenate/7523
  t59/100 -> concatenate/7524
  t59/101 -> concatenate/7525
  t59/102 -> concatenate/7526
  t59/103 -> concatenate/7527
  t59/104 -> concatenate/7528
  t59/105 -> concatenate/7529
  t59/106 -> concatenate/7530
  t59/107 -> concatenate/7531
  t59/108 -> concatenate/7532
  t59/109 -> concatenate/7533
  t59/110 -> concatenate/7534
  t59/111 -> concatenate/7535
  t59/112 -> concatenate/7536
  t59/113 -> concatenate/7537
  t59/114 -> concatenate/7538
  t59/115 -> concatenate/7539
  t59/116 -> concatenate/7540
  t59/117 -> concatenate/7541
  t59/118 -> concatenate/7542
  t59/119 -> concatenate/7543
  t59/120 -> concatenate/7544
  t59/121 -> concatenate/7545
  t59/122 -> concatenate/7546
  t59/123 -> concatenate/7547
  t59/124 -> concatenate/7548
  t59/125 -> concatenate/7549
  t59/126 -> concatenate/7550
  t59/127 -> concatenate/7551
  t59/128 -> concatenate/7552
  t60/1 -> concatenate/7553
  t60/2 -> concatenate/7554
  t60/3 -> concatenate/7555
  t60/4 -> concatenate/7556
  t60/5 -> concatenate/7557
  t60/6 -> concatenate/7558
  t60/7 -> concatenate/7559
  t60/8 -> concatenate/7560
  t60/9 -> concatenate/7561
  t60/10 -> concatenate/7562
  t60/11 -> concatenate/7563
  t60/12 -> concatenate/7564
  t60/13 -> concatenate/7565
  t60/14 -> concatenate/7566
  t60/15 -> concatenate/7567
  t60/16 -> concatenate/7568
  t60/17 -> concatenate/7569
  t60/18 -> concatenate/7570
  t60/19 -> concatenate/7571
  t60/20 -> concatenate/7572
  t60/21 -> concatenate/7573
  t60/22 -> concatenate/7574
  t60/23 -> concatenate/7575
  t60/24 -> concatenate/7576
  t60/25 -> concatenate/7577
  t60/26 -> concatenate/7578
  t60/27 -> concatenate/7579
  t60/28 -> concatenate/7580
  t60/29 -> concatenate/7581
  t60/30 -> concatenate/7582
  t60/31 -> concatenate/7583
  t60/32 -> concatenate/7584
  t60/33 -> concatenate/7585
  t60/34 -> concatenate/7586
  t60/35 -> concatenate/7587
  t60/36 -> concatenate/7588
  t60/37 -> concatenate/7589
  t60/38 -> concatenate/7590
  t60/39 -> concatenate/7591
  t60/40 -> concatenate/7592
  t60/41 -> concatenate/7593
  t60/42 -> concatenate/7594
  t60/43 -> concatenate/7595
  t60/44 -> concatenate/7596
  t60/45 -> concatenate/7597
  t60/46 -> concatenate/7598
  t60/47 -> concatenate/7599
  t60/48 -> concatenate/7600
  t60/49 -> concatenate/7601
  t60/50 -> concatenate/7602
  t60/51 -> concatenate/7603
  t60/52 -> concatenate/7604
  t60/53 -> concatenate/7605
  t60/54 -> concatenate/7606
  t60/55 -> concatenate/7607
  t60/56 -> concatenate/7608
  t60/57 -> concatenate/7609
  t60/58 -> concatenate/7610
  t60/59 -> concatenate/7611
  t60/60 -> concatenate/7612
  t60/61 -> concatenate/7613
  t60/62 -> concatenate/7614
  t60/63 -> concatenate/7615
  t60/64 -> concatenate/7616
  t60/65 -> concatenate/7617
  t60/66 -> concatenate/7618
  t60/67 -> concatenate/7619
  t60/68 -> concatenate/7620
  t60/69 -> concatenate/7621
  t60/70 -> concatenate/7622
  t60/71 -> concatenate/7623
  t60/72 -> concatenate/7624
  t60/73 -> concatenate/7625
  t60/74 -> concatenate/7626
  t60/75 -> concatenate/7627
  t60/76 -> concatenate/7628
  t60/77 -> concatenate/7629
  t60/78 -> concatenate/7630
  t60/79 -> concatenate/7631
  t60/80 -> concatenate/7632
  t60/81 -> concatenate/7633
  t60/82 -> concatenate/7634
  t60/83 -> concatenate/7635
  t60/84 -> concatenate/7636
  t60/85 -> concatenate/7637
  t60/86 -> concatenate/7638
  t60/87 -> concatenate/7639
  t60/88 -> concatenate/7640
  t60/89 -> concatenate/7641
  t60/90 -> concatenate/7642
  t60/91 -> concatenate/7643
  t60/92 -> concatenate/7644
  t60/93 -> concatenate/7645
  t60/94 -> concatenate/7646
  t60/95 -> concatenate/7647
  t60/96 -> concatenate/7648
  t60/97 -> concatenate/7649
  t60/98 -> concatenate/7650
  t60/99 -> concatenate/7651
  t60/100 -> concatenate/7652
  t60/101 -> concatenate/7653
  t60/102 -> concatenate/7654
  t60/103 -> concatenate/7655
  t60/104 -> concatenate/7656
  t60/105 -> concatenate/7657
  t60/106 -> concatenate/7658
  t60/107 -> concatenate/7659
  t60/108 -> concatenate/7660
  t60/109 -> concatenate/7661
  t60/110 -> concatenate/7662
  t60/111 -> concatenate/7663
  t60/112 -> concatenate/7664
  t60/113 -> concatenate/7665
  t60/114 -> concatenate/7666
  t60/115 -> concatenate/7667
  t60/116 -> concatenate/7668
  t60/117 -> concatenate/7669
  t60/118 -> concatenate/7670
  t60/119 -> concatenate/7671
  t60/120 -> concatenate/7672
  t60/121 -> concatenate/7673
  t60/122 -> concatenate/7674
  t60/123 -> concatenate/7675
  t60/124 -> concatenate/7676
  t60/125 -> concatenate/7677
  t60/126 -> concatenate/7678
  t60/127 -> concatenate/7679
  t60/128 -> concatenate/7680
  t61/1 -> concatenate/7681
  t61/2 -> concatenate/7682
  t61/3 -> concatenate/7683
  t61/4 -> concatenate/7684
  t61/5 -> concatenate/7685
  t61/6 -> concatenate/7686
  t61/7 -> concatenate/7687
  t61/8 -> concatenate/7688
  t61/9 -> concatenate/7689
  t61/10 -> concatenate/7690
  t61/11 -> concatenate/7691
  t61/12 -> concatenate/7692
  t61/13 -> concatenate/7693
  t61/14 -> concatenate/7694
  t61/15 -> concatenate/7695
  t61/16 -> concatenate/7696
  t61/17 -> concatenate/7697
  t61/18 -> concatenate/7698
  t61/19 -> concatenate/7699
  t61/20 -> concatenate/7700
  t61/21 -> concatenate/7701
  t61/22 -> concatenate/7702
  t61/23 -> concatenate/7703
  t61/24 -> concatenate/7704
  t61/25 -> concatenate/7705
  t61/26 -> concatenate/7706
  t61/27 -> concatenate/7707
  t61/28 -> concatenate/7708
  t61/29 -> concatenate/7709
  t61/30 -> concatenate/7710
  t61/31 -> concatenate/7711
  t61/32 -> concatenate/7712
  t61/33 -> concatenate/7713
  t61/34 -> concatenate/7714
  t61/35 -> concatenate/7715
  t61/36 -> concatenate/7716
  t61/37 -> concatenate/7717
  t61/38 -> concatenate/7718
  t61/39 -> concatenate/7719
  t61/40 -> concatenate/7720
  t61/41 -> concatenate/7721
  t61/42 -> concatenate/7722
  t61/43 -> concatenate/7723
  t61/44 -> concatenate/7724
  t61/45 -> concatenate/7725
  t61/46 -> concatenate/7726
  t61/47 -> concatenate/7727
  t61/48 -> concatenate/7728
  t61/49 -> concatenate/7729
  t61/50 -> concatenate/7730
  t61/51 -> concatenate/7731
  t61/52 -> concatenate/7732
  t61/53 -> concatenate/7733
  t61/54 -> concatenate/7734
  t61/55 -> concatenate/7735
  t61/56 -> concatenate/7736
  t61/57 -> concatenate/7737
  t61/58 -> concatenate/7738
  t61/59 -> concatenate/7739
  t61/60 -> concatenate/7740
  t61/61 -> concatenate/7741
  t61/62 -> concatenate/7742
  t61/63 -> concatenate/7743
  t61/64 -> concatenate/7744
  t61/65 -> concatenate/7745
  t61/66 -> concatenate/7746
  t61/67 -> concatenate/7747
  t61/68 -> concatenate/7748
  t61/69 -> concatenate/7749
  t61/70 -> concatenate/7750
  t61/71 -> concatenate/7751
  t61/72 -> concatenate/7752
  t61/73 -> concatenate/7753
  t61/74 -> concatenate/7754
  t61/75 -> concatenate/7755
  t61/76 -> concatenate/7756
  t61/77 -> concatenate/7757
  t61/78 -> concatenate/7758
  t61/79 -> concatenate/7759
  t61/80 -> concatenate/7760
  t61/81 -> concatenate/7761
  t61/82 -> concatenate/7762
  t61/83 -> concatenate/7763
  t61/84 -> concatenate/7764
  t61/85 -> concatenate/7765
  t61/86 -> concatenate/7766
  t61/87 -> concatenate/7767
  t61/88 -> concatenate/7768
  t61/89 -> concatenate/7769
  t61/90 -> concatenate/7770
  t61/91 -> concatenate/7771
  t61/92 -> concatenate/7772
  t61/93 -> concatenate/7773
  t61/94 -> concatenate/7774
  t61/95 -> concatenate/7775
  t61/96 -> concatenate/7776
  t61/97 -> concatenate/7777
  t61/98 -> concatenate/7778
  t61/99 -> concatenate/7779
  t61/100 -> concatenate/7780
  t61/101 -> concatenate/7781
  t61/102 -> concatenate/7782
  t61/103 -> concatenate/7783
  t61/104 -> concatenate/7784
  t61/105 -> concatenate/7785
  t61/106 -> concatenate/7786
  t61/107 -> concatenate/7787
  t61/108 -> concatenate/7788
  t61/109 -> concatenate/7789
  t61/110 -> concatenate/7790
  t61/111 -> concatenate/7791
  t61/112 -> concatenate/7792
  t61/113 -> concatenate/7793
  t61/114 -> concatenate/7794
  t61/115 -> concatenate/7795
  t61/116 -> concatenate/7796
  t61/117 -> concatenate/7797
  t61/118 -> concatenate/7798
  t61/119 -> concatenate/7799
  t61/120 -> concatenate/7800
  t61/121 -> concatenate/7801
  t61/122 -> concatenate/7802
  t61/123 -> concatenate/7803
  t61/124 -> concatenate/7804
  t61/125 -> concatenate/7805
  t61/126 -> concatenate/7806
  t61/127 -> concatenate/7807
  t61/128 -> concatenate/7808
  t62/1 -> concatenate/7809
  t62/2 -> concatenate/7810
  t62/3 -> concatenate/7811
  t62/4 -> concatenate/7812
  t62/5 -> concatenate/7813
  t62/6 -> concatenate/7814
  t62/7 -> concatenate/7815
  t62/8 -> concatenate/7816
  t62/9 -> concatenate/7817
  t62/10 -> concatenate/7818
  t62/11 -> concatenate/7819
  t62/12 -> concatenate/7820
  t62/13 -> concatenate/7821
  t62/14 -> concatenate/7822
  t62/15 -> concatenate/7823
  t62/16 -> concatenate/7824
  t62/17 -> concatenate/7825
  t62/18 -> concatenate/7826
  t62/19 -> concatenate/7827
  t62/20 -> concatenate/7828
  t62/21 -> concatenate/7829
  t62/22 -> concatenate/7830
  t62/23 -> concatenate/7831
  t62/24 -> concatenate/7832
  t62/25 -> concatenate/7833
  t62/26 -> concatenate/7834
  t62/27 -> concatenate/7835
  t62/28 -> concatenate/7836
  t62/29 -> concatenate/7837
  t62/30 -> concatenate/7838
  t62/31 -> concatenate/7839
  t62/32 -> concatenate/7840
  t62/33 -> concatenate/7841
  t62/34 -> concatenate/7842
  t62/35 -> concatenate/7843
  t62/36 -> concatenate/7844
  t62/37 -> concatenate/7845
  t62/38 -> concatenate/7846
  t62/39 -> concatenate/7847
  t62/40 -> concatenate/7848
  t62/41 -> concatenate/7849
  t62/42 -> concatenate/7850
  t62/43 -> concatenate/7851
  t62/44 -> concatenate/7852
  t62/45 -> concatenate/7853
  t62/46 -> concatenate/7854
  t62/47 -> concatenate/7855
  t62/48 -> concatenate/7856
  t62/49 -> concatenate/7857
  t62/50 -> concatenate/7858
  t62/51 -> concatenate/7859
  t62/52 -> concatenate/7860
  t62/53 -> concatenate/7861
  t62/54 -> concatenate/7862
  t62/55 -> concatenate/7863
  t62/56 -> concatenate/7864
  t62/57 -> concatenate/7865
  t62/58 -> concatenate/7866
  t62/59 -> concatenate/7867
  t62/60 -> concatenate/7868
  t62/61 -> concatenate/7869
  t62/62 -> concatenate/7870
  t62/63 -> concatenate/7871
  t62/64 -> concatenate/7872
  t62/65 -> concatenate/7873
  t62/66 -> concatenate/7874
  t62/67 -> concatenate/7875
  t62/68 -> concatenate/7876
  t62/69 -> concatenate/7877
  t62/70 -> concatenate/7878
  t62/71 -> concatenate/7879
  t62/72 -> concatenate/7880
  t62/73 -> concatenate/7881
  t62/74 -> concatenate/7882
  t62/75 -> concatenate/7883
  t62/76 -> concatenate/7884
  t62/77 -> concatenate/7885
  t62/78 -> concatenate/7886
  t62/79 -> concatenate/7887
  t62/80 -> concatenate/7888
  t62/81 -> concatenate/7889
  t62/82 -> concatenate/7890
  t62/83 -> concatenate/7891
  t62/84 -> concatenate/7892
  t62/85 -> concatenate/7893
  t62/86 -> concatenate/7894
  t62/87 -> concatenate/7895
  t62/88 -> concatenate/7896
  t62/89 -> concatenate/7897
  t62/90 -> concatenate/7898
  t62/91 -> concatenate/7899
  t62/92 -> concatenate/7900
  t62/93 -> concatenate/7901
  t62/94 -> concatenate/7902
  t62/95 -> concatenate/7903
  t62/96 -> concatenate/7904
  t62/97 -> concatenate/7905
  t62/98 -> concatenate/7906
  t62/99 -> concatenate/7907
  t62/100 -> concatenate/7908
  t62/101 -> concatenate/7909
  t62/102 -> concatenate/7910
  t62/103 -> concatenate/7911
  t62/104 -> concatenate/7912
  t62/105 -> concatenate/7913
  t62/106 -> concatenate/7914
  t62/107 -> concatenate/7915
  t62/108 -> concatenate/7916
  t62/109 -> concatenate/7917
  t62/110 -> concatenate/7918
  t62/111 -> concatenate/7919
  t62/112 -> concatenate/7920
  t62/113 -> concatenate/7921
  t62/114 -> concatenate/7922
  t62/115 -> concatenate/7923
  t62/116 -> concatenate/7924
  t62/117 -> concatenate/7925
  t62/118 -> concatenate/7926
  t62/119 -> concatenate/7927
  t62/120 -> concatenate/7928
  t62/121 -> concatenate/7929
  t62/122 -> concatenate/7930
  t62/123 -> concatenate/7931
  t62/124 -> concatenate/7932
  t62/125 -> concatenate/7933
  t62/126 -> concatenate/7934
  t62/127 -> concatenate/7935
  t62/128 -> concatenate/7936
  t63/1 -> concatenate/7937
  t63/2 -> concatenate/7938
  t63/3 -> concatenate/7939
  t63/4 -> concatenate/7940
  t63/5 -> concatenate/7941
  t63/6 -> concatenate/7942
  t63/7 -> concatenate/7943
  t63/8 -> concatenate/7944
  t63/9 -> concatenate/7945
  t63/10 -> concatenate/7946
  t63/11 -> concatenate/7947
  t63/12 -> concatenate/7948
  t63/13 -> concatenate/7949
  t63/14 -> concatenate/7950
  t63/15 -> concatenate/7951
  t63/16 -> concatenate/7952
  t63/17 -> concatenate/7953
  t63/18 -> concatenate/7954
  t63/19 -> concatenate/7955
  t63/20 -> concatenate/7956
  t63/21 -> concatenate/7957
  t63/22 -> concatenate/7958
  t63/23 -> concatenate/7959
  t63/24 -> concatenate/7960
  t63/25 -> concatenate/7961
  t63/26 -> concatenate/7962
  t63/27 -> concatenate/7963
  t63/28 -> concatenate/7964
  t63/29 -> concatenate/7965
  t63/30 -> concatenate/7966
  t63/31 -> concatenate/7967
  t63/32 -> concatenate/7968
  t63/33 -> concatenate/7969
  t63/34 -> concatenate/7970
  t63/35 -> concatenate/7971
  t63/36 -> concatenate/7972
  t63/37 -> concatenate/7973
  t63/38 -> concatenate/7974
  t63/39 -> concatenate/7975
  t63/40 -> concatenate/7976
  t63/41 -> concatenate/7977
  t63/42 -> concatenate/7978
  t63/43 -> concatenate/7979
  t63/44 -> concatenate/7980
  t63/45 -> concatenate/7981
  t63/46 -> concatenate/7982
  t63/47 -> concatenate/7983
  t63/48 -> concatenate/7984
  t63/49 -> concatenate/7985
  t63/50 -> concatenate/7986
  t63/51 -> concatenate/7987
  t63/52 -> concatenate/7988
  t63/53 -> concatenate/7989
  t63/54 -> concatenate/7990
  t63/55 -> concatenate/7991
  t63/56 -> concatenate/7992
  t63/57 -> concatenate/7993
  t63/58 -> concatenate/7994
  t63/59 -> concatenate/7995
  t63/60 -> concatenate/7996
  t63/61 -> concatenate/7997
  t63/62 -> concatenate/7998
  t63/63 -> concatenate/7999
  t63/64 -> concatenate/8000
  t63/65 -> concatenate/8001
  t63/66 -> concatenate/8002
  t63/67 -> concatenate/8003
  t63/68 -> concatenate/8004
  t63/69 -> concatenate/8005
  t63/70 -> concatenate/8006
  t63/71 -> concatenate/8007
  t63/72 -> concatenate/8008
  t63/73 -> concatenate/8009
  t63/74 -> concatenate/8010
  t63/75 -> concatenate/8011
  t63/76 -> concatenate/8012
  t63/77 -> concatenate/8013
  t63/78 -> concatenate/8014
  t63/79 -> concatenate/8015
  t63/80 -> concatenate/8016
  t63/81 -> concatenate/8017
  t63/82 -> concatenate/8018
  t63/83 -> concatenate/8019
  t63/84 -> concatenate/8020
  t63/85 -> concatenate/8021
  t63/86 -> concatenate/8022
  t63/87 -> concatenate/8023
  t63/88 -> concatenate/8024
  t63/89 -> concatenate/8025
  t63/90 -> concatenate/8026
  t63/91 -> concatenate/8027
  t63/92 -> concatenate/8028
  t63/93 -> concatenate/8029
  t63/94 -> concatenate/8030
  t63/95 -> concatenate/8031
  t63/96 -> concatenate/8032
  t63/97 -> concatenate/8033
  t63/98 -> concatenate/8034
  t63/99 -> concatenate/8035
  t63/100 -> concatenate/8036
  t63/101 -> concatenate/8037
  t63/102 -> concatenate/8038
  t63/103 -> concatenate/8039
  t63/104 -> concatenate/8040
  t63/105 -> concatenate/8041
  t63/106 -> concatenate/8042
  t63/107 -> concatenate/8043
  t63/108 -> concatenate/8044
  t63/109 -> concatenate/8045
  t63/110 -> concatenate/8046
  t63/111 -> concatenate/8047
  t63/112 -> concatenate/8048
  t63/113 -> concatenate/8049
  t63/114 -> concatenate/8050
  t63/115 -> concatenate/8051
  t63/116 -> concatenate/8052
  t63/117 -> concatenate/8053
  t63/118 -> concatenate/8054
  t63/119 -> concatenate/8055
  t63/120 -> concatenate/8056
  t63/121 -> concatenate/8057
  t63/122 -> concatenate/8058
  t63/123 -> concatenate/8059
  t63/124 -> concatenate/8060
  t63/125 -> concatenate/8061
  t63/126 -> concatenate/8062
  t63/127 -> concatenate/8063
  t63/128 -> concatenate/8064
  t64/1 -> concatenate/8065
  t64/2 -> concatenate/8066
  t64/3 -> concatenate/8067
  t64/4 -> concatenate/8068
  t64/5 -> concatenate/8069
  t64/6 -> concatenate/8070
  t64/7 -> concatenate/8071
  t64/8 -> concatenate/8072
  t64/9 -> concatenate/8073
  t64/10 -> concatenate/8074
  t64/11 -> concatenate/8075
  t64/12 -> concatenate/8076
  t64/13 -> concatenate/8077
  t64/14 -> concatenate/8078
  t64/15 -> concatenate/8079
  t64/16 -> concatenate/8080
  t64/17 -> concatenate/8081
  t64/18 -> concatenate/8082
  t64/19 -> concatenate/8083
  t64/20 -> concatenate/8084
  t64/21 -> concatenate/8085
  t64/22 -> concatenate/8086
  t64/23 -> concatenate/8087
  t64/24 -> concatenate/8088
  t64/25 -> concatenate/8089
  t64/26 -> concatenate/8090
  t64/27 -> concatenate/8091
  t64/28 -> concatenate/8092
  t64/29 -> concatenate/8093
  t64/30 -> concatenate/8094
  t64/31 -> concatenate/8095
  t64/32 -> concatenate/8096
  t64/33 -> concatenate/8097
  t64/34 -> concatenate/8098
  t64/35 -> concatenate/8099
  t64/36 -> concatenate/8100
  t64/37 -> concatenate/8101
  t64/38 -> concatenate/8102
  t64/39 -> concatenate/8103
  t64/40 -> concatenate/8104
  t64/41 -> concatenate/8105
  t64/42 -> concatenate/8106
  t64/43 -> concatenate/8107
  t64/44 -> concatenate/8108
  t64/45 -> concatenate/8109
  t64/46 -> concatenate/8110
  t64/47 -> concatenate/8111
  t64/48 -> concatenate/8112
  t64/49 -> concatenate/8113
  t64/50 -> concatenate/8114
  t64/51 -> concatenate/8115
  t64/52 -> concatenate/8116
  t64/53 -> concatenate/8117
  t64/54 -> concatenate/8118
  t64/55 -> concatenate/8119
  t64/56 -> concatenate/8120
  t64/57 -> concatenate/8121
  t64/58 -> concatenate/8122
  t64/59 -> concatenate/8123
  t64/60 -> concatenate/8124
  t64/61 -> concatenate/8125
  t64/62 -> concatenate/8126
  t64/63 -> concatenate/8127
  t64/64 -> concatenate/8128
  t64/65 -> concatenate/8129
  t64/66 -> concatenate/8130
  t64/67 -> concatenate/8131
  t64/68 -> concatenate/8132
  t64/69 -> concatenate/8133
  t64/70 -> concatenate/8134
  t64/71 -> concatenate/8135
  t64/72 -> concatenate/8136
  t64/73 -> concatenate/8137
  t64/74 -> concatenate/8138
  t64/75 -> concatenate/8139
  t64/76 -> concatenate/8140
  t64/77 -> concatenate/8141
  t64/78 -> concatenate/8142
  t64/79 -> concatenate/8143
  t64/80 -> concatenate/8144
  t64/81 -> concatenate/8145
  t64/82 -> concatenate/8146
  t64/83 -> concatenate/8147
  t64/84 -> concatenate/8148
  t64/85 -> concatenate/8149
  t64/86 -> concatenate/8150
  t64/87 -> concatenate/8151
  t64/88 -> concatenate/8152
  t64/89 -> concatenate/8153
  t64/90 -> concatenate/8154
  t64/91 -> concatenate/8155
  t64/92 -> concatenate/8156
  t64/93 -> concatenate/8157
  t64/94 -> concatenate/8158
  t64/95 -> concatenate/8159
  t64/96 -> concatenate/8160
  t64/97 -> concatenate/8161
  t64/98 -> concatenate/8162
  t64/99 -> concatenate/8163
  t64/100 -> concatenate/8164
  t64/101 -> concatenate/8165
  t64/102 -> concatenate/8166
  t64/103 -> concatenate/8167
  t64/104 -> concatenate/8168
  t64/105 -> concatenate/8169
  t64/106 -> concatenate/8170
  t64/107 -> concatenate/8171
  t64/108 -> concatenate/8172
  t64/109 -> concatenate/8173
  t64/110 -> concatenate/8174
  t64/111 -> concatenate/8175
  t64/112 -> concatenate/8176
  t64/113 -> concatenate/8177
  t64/114 -> concatenate/8178
  t64/115 -> concatenate/8179
  t64/116 -> concatenate/8180
  t64/117 -> concatenate/8181
  t64/118 -> concatenate/8182
  t64/119 -> concatenate/8183
  t64/120 -> concatenate/8184
  t64/121 -> concatenate/8185
  t64/122 -> concatenate/8186
  t64/123 -> concatenate/8187
  t64/124 -> concatenate/8188
  t64/125 -> concatenate/8189
  t64/126 -> concatenate/8190
  t64/127 -> concatenate/8191
  t64/128 -> concatenate/8192
